simulink model "RefModel_Task"  (R2020a)
settings: Solver=ode1  StartTime=0.0  StopTime=10.0  FixedStep=Ts_Task.Ts_base  RelTol=1e-3
undefined symbols (not defined in the file or in its folder): groundspeedCmd, heightCmd, rollCmd
(part 2 of 5)

== stateflow chart RefModel_Task/Task_StateFlow ==
  state LogData [parallel]
    en:
    settings: executionOrder=17
    state Work
      en,du:
      du_func;
    (default) -> LogData.Work
  state ParserInput [parallel]
    en:
    initPathModeOut;
    initWindParam;
    updateInput;
    enterNum_Land = 0;
    du:
    % ComFlightOut = updateInput;
    updateInput;
    updatePathModeOut;
    % 计算有效航路点数
    PathModeOut.validPathNum = calValidPointNum;
    % 姿态是否稳定
    isAttitudeStable_globalvar = isAttitudeStable;
    % 更新当前航点
    updatePreAndCurPathPoint;
    % on every(300, tick): isPathDataValid;
    settings: executionOrder=1
  state ParserCmd [parallel]
    % 处理Mavlink指令
    en:
    printComInfo('TaskModel Start!!!!',0)
    initInputCmdParam
    du:
    du_func_cmd;
    du_func_singleMode;
    settings: executionOrder=2
    state REMOTE [parallel]
      settings: executionOrder=1
      state Manual
        en:
        manual_du_func
      state Auto
        en:
        auto_du_func
      (default) -> Manual
      Manual -> Auto [order 1] : [IN_MAV.remote_control_t.chG_Mag < 1500]
      Manual -> Auto [order 2] : [TaskParam.getOutOfRemote]
      Auto -> Manual : [IN_MAV.remote_control_t.chG_Mag >= 1500 && ...
          | ~TaskParam.getOutOfRemote]
  state BreakPoint [parallel]
    settings: executionOrder=18
    state BeforePath
      en,du:
    state InPath
      en,du:
    state PauseInPath
      en,du:
    state InGoHome
      en:
      en_func;
    (default) -> BeforePath
    (junction 2115) -> BeforePath
    (junction 2112) -> (junction 2115)
    BeforePath -> InPath : [PathModeOut.flightTaskMode == ENUM_FlightTaskMode.PathFollowMode]
    InPath -> PauseInPath [order 2] : [PathModeOut.flightTaskMode == ENUM_FlightTaskMode.AirStandByMode]
    PauseInPath -> InPath [order 1] : [PathModeOut.flightTaskMode == ENUM_FlightTaskMode.PathFollowMode]
    InPath -> (junction 2121) [order 1]
    PauseInPath -> (junction 2124) [order 2]
    (junction 2124) -> (junction 2121)
    (junction 2121) -> InGoHome : [PathModeOut.flightTaskMode == ENUM_FlightTaskMode.GoHomeMode || ...
        | PathModeOut.flightTaskMode == ENUM_FlightTaskMode.Fix2Rotor_Mode]
    InGoHome -> (junction 2112) : [PathModeOut.flightTaskMode == ENUM_FlightTaskMode.GroundStandByMode]
  state PowerConsumer [parallel]
    settings: executionOrder=3
    state Work
      en,du:
      du_func;
    (default) -> PowerConsumer.Work
  state PrintfCriticalInfo [parallel]
    on every(120,tick): info_60tick();
    settings: executionOrder=4
  state FLIGHTMODE [parallel]
    settings: executionOrder=5
    state AUTO_TASK
      en:
      % 进入模式
      printDebugInfo('AUTOTASK','Enter',1)
      RTInfo.Task = ENUM_RTInfo_Task.Enter_AutoMode; % 更新RT信息
      isAutoMode_globalvar = true;
      PathModeOut.AutoManualMode = ENUM_ControlMode.Auto;
      du:
      du_AUTO_TASK_func;
      ex:
      % 退出模式
      printDebugInfo('AUTOTASK','Exit',1)
      state INIT
        en:
        % 进入模式
        printDebugInfo('INIT','Enter')
        RTInfo.Task = ENUM_RTInfo_Task.Enter_AutoMode_Init; % 更新RT信息
        sendEventWhileEnterAuto
        ex:
        % 退出模式
        printDebugInfo('INIT','Exit')
      state MODE_GOURNDSTANDBY
        en:
        % 进入模式
        printDebugInfo('GroundStandBy','Enter')
        RTInfo.Task = ENUM_RTInfo_Task.Enter_AutoMode_GroundStandBy; % 更新RT信息
        updateLogDataBuffer(ENUM_TaskLogBlockName.TASKLOG_FlightMode,RTInfo.Task,'write'); % 更新log缓存
        PathModeOut.whereIsUAV = ENUM_Where.OnGround;
        hasTaskStarted_globalbar = false;
        ex:
        % 退出模式
        printDebugInfo('GroundStandBy','Exit')
        preTaskMode = ENUM_FlightTaskMode.GroundStandByMode;
        PathModeOut.numTakeOff = PathModeOut.numTakeOff + 1;
        state INIT
          en:
          RTInfo.Task = ENUM_RTInfo_Task.Enter_AutoMode_GroundStandBy_Init; % 更新RT信息
          updateLogDataBuffer(ENUM_TaskLogBlockName.TASKLOG_FlightMode,RTInfo.Task,'write'); % 更新log缓存
          PathModeOut.uavMode = TaskParam.uavMode_InGroundStandByMode;
          PathModeOut.flightTaskMode = ENUM_FlightTaskMode.GroundStandByMode;
          if ~hasTakeOff %  起飞前的地面怠速
          PathModeOut.flightControlMode = ENUM_FlightControlMode.GroundStandByControlMode;
          else % 降落后发动机关车
          PathModeOut.flightControlMode = ENUM_FlightControlMode.RotorShutDown;
          end
          du:
        state TOGO
          en:
          printDebugInfo('GroundStandBy','ToGo')
          RTInfo.Task = ENUM_RTInfo_Task.Enter_AutoMode_GroundStandBy_ToGo; % 更新RT信息
          updateLogDataBuffer(ENUM_TaskLogBlockName.TASKLOG_FlightMode,RTInfo.Task,'write'); % 更新log缓存
          PathModeOut.headingCmd = double(ComFlightOut.curEuler(1));
          du:
          % 实时更新当前航向，避免航向测量修正对起飞模式控制的影响
          PathModeOut.groundspeedCmd = 0;
          % PathModeOut.turnRadiusCmd = 0;
          PathModeOut.heightCmd = 0;
          % 设置侧偏距为0
          PathModeOut.dz = 0;
          % 设置预置滚转
          PathModeOut.rollCmd = 0;
          % 悬停位置
          PathModeOut.turnCenterLL = ComFlightOut.curLLA(1:2);
        (default) -> FLIGHTMODE.AUTO_TASK.MODE_GOURNDSTANDBY.INIT
        FLIGHTMODE.AUTO_TASK.MODE_GOURNDSTANDBY.INIT -> FLIGHTMODE.AUTO_TASK.MODE_GOURNDSTANDBY.TOGO : [isReadyToGo]
      state MODE_TAKEOFF
        en:
        % 进入模式
        printDebugInfo('TakeOff','Enter')
        RTInfo.Task = ENUM_RTInfo_Task.Enter_AutoMode_TakeOff; % 更新RT信息
        updateLogDataBuffer(ENUM_TaskLogBlockName.TASKLOG_FlightMode,RTInfo.Task,'write'); % 更新log缓存
        PathModeOut.whereIsUAV = ENUM_Where.InTheAir;
        hasTakeOff = true;
        du:
        ex:
        % 退出模式
        printDebugInfo('TakeOff','Exit')
        preTaskMode = ENUM_FlightTaskMode.TakeOffMode;
        state INIT
          en:
          RTInfo.Task = ENUM_RTInfo_Task.Enter_AutoMode_TakeOff_Init; % 更新RT信息
          updateLogDataBuffer(ENUM_TaskLogBlockName.TASKLOG_FlightMode,RTInfo.Task,'write'); % 更新log缓存
          PathModeOut.uavMode = TaskParam.uavMode_InTakeOffMode;
          PathModeOut.flightTaskMode = ENUM_FlightTaskMode.TakeOffMode;
          PathModeOut.flightControlMode = ENUM_FlightControlMode.RotorGoUpDownBySpeed;
          % 需计算指令： 高度 航向 速度
          tempIdx = idxStartPathPoint;
          if isPathDataValid && PathModeOut.typeAutoMode == ENUM_AutoModeType.AutoProfile
          % 自动任务模式下
          printDebugInfo('TakeOff','AutoProfile Yes')
          % 航向捕获当前航向
          PathModeOut.headingCmd = double(ComFlightOut.curEuler(1));
          else
          printDebugInfo('TakeOff','AutoProfile No')
          % 航向捕获当前航向
          PathModeOut.headingCmd = double(ComFlightOut.curEuler(1));
          end
          PathModeOut.groundspeedCmd = TaskParam.cruiseSpeed_rotorMode;
          % 设置侧偏距为0
          PathModeOut.dz = 0;
          % 设置预置滚转
          PathModeOut.rollCmd = 0;
          % 悬停位置
          PathModeOut.turnCenterLL = ComFlightOut.curLLA(1:2);
        state DOING_NearGround
          en:
          printDebugInfo('TakeOff','NearGround')
          RTInfo.Task = ENUM_RTInfo_Task.Enter_AutoMode_TakeOff_NearGround; % 更新RT信息
          updateLogDataBuffer(ENUM_TaskLogBlockName.TASKLOG_FlightMode,RTInfo.Task,'write'); % 更新log缓存
          PathModeOut.flightControlMode = ENUM_FlightControlMode.RotorGoUpDownBySpeed;
          PathModeOut.heightCmd = TaskParam.midHeight_TakeOffandLand;
          PathModeOut.maxClimbSpeed = TaskParam.maxClimbSpeed_nearGround_TakeOffandLand;
        state WAITING
          en:
          printDebugInfo('TakeOff','Waiting')
          RTInfo.Task = ENUM_RTInfo_Task.Enter_AutoMode_TakeOff_Waiting; % 更新RT信息
          updateLogDataBuffer(ENUM_TaskLogBlockName.TASKLOG_FlightMode,RTInfo.Task,'write'); % 更新log缓存
          PathModeOut.flightControlMode = ENUM_FlightControlMode.SpotHoverMode;
          PathModeOut.heightCmd = TaskParam.midHeight_TakeOffandLand;
        state DOING_FarGround
          en:
          printDebugInfo('TakeOff','FarGround')
          RTInfo.Task = ENUM_RTInfo_Task.Enter_AutoMode_TakeOff_FarGround; % 更新RT信息
          updateLogDataBuffer(ENUM_TaskLogBlockName.TASKLOG_FlightMode,RTInfo.Task,'write'); % 更新log缓存
          PathModeOut.flightControlMode = ENUM_FlightControlMode.RotorGoUpDownBySpeed;
          PathModeOut.heightCmd = CmdParam_altitude;
          PathModeOut.maxClimbSpeed = TaskParam.maxClimbSpeed_normal_TakeOffandLand+0.5;
        state TOGO
          en:
          printDebugInfo('TakeOff','ToGo')
          RTInfo.Task = ENUM_RTInfo_Task.Enter_AutoMode_TakeOff_ToGo; % 更新RT信息
          updateLogDataBuffer(ENUM_TaskLogBlockName.TASKLOG_FlightMode,RTInfo.Task,'write'); % 更新log缓存
          du:
          % 无条件转入后续模式
          headingMode = 1;
          nextMode = ENUM_FlightTaskMode.Rotor2Fix_Mode ;
          SendEvent_autoGoToNextMode
        state StopHere
          en:
          printDebugInfo('TakeOff','StopHere')
          RTInfo.Task = ENUM_RTInfo_Task.SingleMode_TakeOff_StopHere; % 更新RT信息
          updateLogDataBuffer(ENUM_TaskLogBlockName.TASKLOG_FlightMode,RTInfo.Task,'write'); % 更新log缓存
          du:
        (default) -> FLIGHTMODE.AUTO_TASK.MODE_TAKEOFF.INIT
        FLIGHTMODE.AUTO_TASK.MODE_TAKEOFF.INIT -> (junction 1490)
        (junction 1490) -> DOING_NearGround [order 1] : [hasTaskStarted_globalbar == false]% && ...
            | %ComFlightOut.curLLA(3)<AlgoParams.midHeight_TakeOffandLand+10]
        (junction 1490) -> DOING_FarGround [order 2]
        DOING_NearGround -> WAITING : [hasReachHeight(2)  && isAttitudeStable_globalvar]
        WAITING -> DOING_FarGround : event_startTaskFromAir
            | {hasTaskStarted_globalbar = true;}
        DOING_FarGround -> (junction 2190)
        (junction 2190) -> (junction 2193) [order 1] : [isSingleModeRun]
        (junction 2193) -> FLIGHTMODE.AUTO_TASK.MODE_TAKEOFF.StopHere
        (junction 2190) -> FLIGHTMODE.AUTO_TASK.MODE_TAKEOFF.TOGO [order 2] : [hasReachHeight(2)  && isAttitudeStable_Alevel && after(3,sec) || ...
            | hasReachHeight(5)  && after(5,sec)]
      state MODE_HOVERADJUST
        en:
        % 进入模式
        printDebugInfo('HoverAdjust','Enter')
        HeightCmdBeforeAirStandBy = PathModeOut.heightCmd;
        TaskModeBeforeAirStandBy = preTaskMode;
        HeadingCmdBeforeAirStandBy = PathModeOut.headingCmd;
        PathModeOut.whereIsUAV = ENUM_Where.InTheAir;
        on event_homeChanged: % 着陆过程中暂停时,若home点改变，则继续任务时先gohome
        if (preTaskMode == ENUM_FlightTaskMode.LandMode)  && ...
        PathModeOut.typeAutoMode == ENUM_AutoModeType.SuspendTaskToLand;
        TaskModeBeforeAirStandBy = ENUM_FlightTaskMode.GoHomeMode;
        PathModeOut.typeAutoMode = ENUM_AutoModeType.SuspendTaskToHomeThenLand;
        end
        ex:
        % 退出模式
        printDebugInfo('HoverAdjust','Exit')
        state INIT
          en:
          en_func;
        state WORK
          state DOING
            en:
            en_func;
            du:
            responseManualMove;
          state TOGO
            en:
            printDebugInfo('HoverAdjust','ToGo')
            RTInfo.Task = ENUM_RTInfo_Task.Enter_AutoMode_HoverAdjust_ToGo; % 更新RT信息
            updateLogDataBuffer(ENUM_TaskLogBlockName.TASKLOG_FlightMode,RTInfo.Task,'write'); % 更新log缓存
            switch PathModeOut.typeAutoMode
            case ENUM_AutoModeType.AutoProfile
            RTInfo.Task = ENUM_RTInfo_Task.If_AutoMode_HoverAdjust_ToGo_AutoProfile_Yes; % 更新RT信息
            updateLogDataBuffer(ENUM_TaskLogBlockName.TASKLOG_FlightMode,RTInfo.Task,'write'); % 更新log缓存
            SendEvent_autoGoToNextMode
            case  {ENUM_AutoModeType.SuspendTaskToLand,...
            ENUM_AutoModeType.Fix2Rotor2Home2Land}
            nextMode = ENUM_FlightTaskMode.LandMode;
            SendEvent_autoGoToNextMode
            case ENUM_AutoModeType.SuspendTaskToHome
            case ENUM_AutoModeType.Fix2Rotor2HoverAdjust
            case ENUM_AutoModeType.SuspendTaskToHomeThenLand
            nextMode = ENUM_FlightTaskMode.LandMode;
            SendEvent_autoGoToNextMode
            case ENUM_AutoModeType.PauseInAir
            PathModeOut.typeAutoMode = typeAutoModePre;
            send(event_gotoWaitForContinue,FLIGHTMODE.AUTO_TASK)
            otherwise
            % 保持在当前模式
            end
            du:
            responseManualMove;
          state WaitForContinue
            en:
            printDebugInfo('HoverAdjust','WaitForContinue')
            RTInfo.Task = ENUM_RTInfo_Task.Enter_AutoMode_HoverAdjust_WaitForContinue; % 更新RT信息
            updateLogDataBuffer(ENUM_TaskLogBlockName.TASKLOG_FlightMode,RTInfo.Task,'write'); % 更新log缓存
            du:
            responseManualMove;
          FLIGHTMODE.AUTO_TASK.MODE_HOVERADJUST.WORK.DOING -> (junction 1747) [order 2] : event_gotoWaitForContinue
          FLIGHTMODE.AUTO_TASK.MODE_HOVERADJUST.WORK.DOING -> FLIGHTMODE.AUTO_TASK.MODE_HOVERADJUST.WORK.TOGO [order 1] : [(hasMatchAllConditons && isAttitudeStable_globalvar && after(ceil(6/Ts),tick) && nextMode ~= ENUM_FlightTaskMode.LandMode) || ...
              | (hasReachLatLon_assign(10) && hasReachHeight && isAttitudeStable_globalvar &&  after(ceil(30/Ts),tick) && nextMode ~= ENUM_FlightTaskMode.LandMode) || ...
              | (hasReachLatLon_assign(2) && hasReachHeight && isAttitudeStable_Alevel && after(ceil(6/Ts),tick) && nextMode == ENUM_FlightTaskMode.LandMode) || ...
              | (isAttitudeStable_globalvar && after(ceil(4/Ts),tick) && PathModeOut.typeAutoMode == ENUM_AutoModeType.SuspendTaskToLand)]
          FLIGHTMODE.AUTO_TASK.MODE_HOVERADJUST.WORK.TOGO -> WaitForContinue : event_gotoWaitForContinue
          (junction 1747) -> WaitForContinue
        state StopHere
          en:
          printDebugInfo('HovverAdjust','StopHere')
          RTInfo.Task = ENUM_RTInfo_Task.SingleMode_HovverAdjust_StopHere; % 更新RT信息
          updateLogDataBuffer(ENUM_TaskLogBlockName.TASKLOG_FlightMode,RTInfo.Task,'write'); % 更新log缓存
          du:
        state ExitFromContinue
          en:
          printDebugInfo('HoverAdjust','Enter ExitFromContinue')
          RTInfo.Task = ENUM_RTInfo_Task.Enter_AutoMode_HoverAdjust_ExitFromContinue; % 更新RT信息
          updateLogDataBuffer(ENUM_TaskLogBlockName.TASKLOG_FlightMode,RTInfo.Task,'write'); % 更新log缓存
          SendEvent_ContinueFromPause
          du:
          SendEvent_ContinueFromPause
        (default) -> FLIGHTMODE.AUTO_TASK.MODE_HOVERADJUST.INIT
        FLIGHTMODE.AUTO_TASK.MODE_HOVERADJUST.INIT -> FLIGHTMODE.AUTO_TASK.MODE_HOVERADJUST.WORK.DOING : [isReadyToGo]
        WaitForContinue -> (junction 2199)
        (junction 2199) -> (junction 2197) [order 1] : [isSingleModeRun]
        (junction 2199) -> FLIGHTMODE.AUTO_TASK.MODE_HOVERADJUST.ExitFromContinue [order 2] : manual_continueProfile || ...
            | event_startTaskFromAir % 起飞前半段
        (junction 2197) -> FLIGHTMODE.AUTO_TASK.MODE_HOVERADJUST.StopHere
      state MODE_ROTOR2FIX
        en:
        % 进入模式
        printDebugInfo('Rotor2Fix','Enter')
        RTInfo.Task = ENUM_RTInfo_Task.Enter_AutoMode_Rotor2Fix; % 更新RT信息
        updateLogDataBuffer(ENUM_TaskLogBlockName.TASKLOG_FlightMode,RTInfo.Task,'write'); % 更新log缓存
        PathModeOut.whereIsUAV = ENUM_Where.InTheAir;
        ex:
        % 退出模式
        printDebugInfo('Rotor2Fix','Exit')
        preTaskMode = ENUM_FlightTaskMode.Rotor2Fix_Mode;
        % PathModeOut.uavMode = ENUM_UAVMode.Fix; % 防止该模
        state INIT
          en:
          printDebugInfo('Rotor2Fix','Init')
          RTInfo.Task = ENUM_RTInfo_Task.Enter_AutoMode_Rotor2Fix_Init; % 更新RT信息
          updateLogDataBuffer(ENUM_TaskLogBlockName.TASKLOG_FlightMode,RTInfo.Task,'write'); % 更新log缓存
          PathModeOut.uavMode = TaskParam.uavMode_InRotor2FixMode;
          PathModeOut.flightTaskMode = ENUM_FlightTaskMode.Rotor2Fix_Mode;
          PathModeOut.flightControlMode = ENUM_FlightControlMode.HeightKeepMode;
          % 需计算指令： 高度 航向 速度
          tempIdx = idxStartPathPoint;
          if isPathDataValid && PathModeOut.typeAutoMode == ENUM_AutoModeType.AutoProfile
          printDebugInfo('Rotor2Fix','AutoProfile Yes')
          RTInfo.Task = ENUM_RTInfo_Task.If_AutoMode_Rotor2Fix_Init_AutoProfile_Yes; % 更新RT信息
          updateLogDataBuffer(ENUM_TaskLogBlockName.TASKLOG_FlightMode,RTInfo.Task,'write'); % 更新log缓存
          % 自动任务模式下
          % 高度指令延续前一模式
          % 航向指令延续前一模式
          PathModeOut.groundspeedCmd = TaskParam.cruiseSpeed_cruise;
          else
          printDebugInfo('Rotor2Fix','AutoProfile No')
          % 手动选择该模式
          % 捕获当前高度
          PathModeOut.heightCmd = double(ComFlightOut.curLLA(3));
          % 捕获当前速度,设定最小值
          PathModeOut.groundspeedCmd = max(TaskParam.cruiseSpeed_cruise,ComFlightOut.curGroundSpeed);
          end
          % 捕获当前航向
          PathModeOut.headingCmd = double(ComFlightOut.curEuler(1));
          % 设置侧偏距为0
          PathModeOut.dz = 0;
          % 设置预置滚转
          PathModeOut.rollCmd = 0;
          % 最大爬升率
          PathModeOut.maxClimbSpeed = TaskParam.maxClimbSpeed_fixMode;
        state TOGO
          en:
          printDebugInfo('Rotor2Fix','ToGo')
          RTInfo.Task = ENUM_RTInfo_Task.Enter_AutoMode_Rotor2Fix_ToGo; % 更新RT信息
          updateLogDataBuffer(ENUM_TaskLogBlockName.TASKLOG_FlightMode,RTInfo.Task,'write'); % 更新log缓存
          PathModeOut.uavMode = ENUM_UAVMode.Fix;
          du:
          switch PathModeOut.typeAutoMode
          case ENUM_AutoModeType.AutoProfile
          printDebugInfo('Rotor2Fix','Switch AutoProfile')
          RTInfo.Task = ENUM_RTInfo_Task.If_AutoMode_Rotor2Fix_ToGo_AutoProfile_Yes; % 更新RT信息
          updateLogDataBuffer(ENUM_TaskLogBlockName.TASKLOG_FlightMode,RTInfo.Task,'write'); % 更新log缓存
          SendEvent_autoGoToNextMode
          case {ENUM_AutoModeType.SuspendTaskToHomeThenLand,ENUM_AutoModeType.SuspendTaskToHome}
          printDebugInfo('Rotor2Fix','Switch Fix2Rotor2Home2Land')
          RTInfo.Task = ENUM_RTInfo_Task.If_AutoMode_Rotor2Fix_ToGo_Fix2Rotor2Home2Land_Yes; % 更新RT信息
          updateLogDataBuffer(ENUM_TaskLogBlockName.TASKLOG_FlightMode,RTInfo.Task,'write'); % 更新log缓存
          send(event_fix2Rotor2Home2Land,FLIGHTMODE.AUTO_TASK);
          case ENUM_AutoModeType.SuspendTaskToLand
          printDebugInfo('Rotor2Fix','Switch SuspendTaskToLand')
          RTInfo.Task = ENUM_RTInfo_Task.If_AutoMode_Rotor2Fix_ToGo_SuspendTaskToLand_Yes; % 更新RT信息
          updateLogDataBuffer(ENUM_TaskLogBlockName.TASKLOG_FlightMode,RTInfo.Task,'write'); % 更新log缓存
          send(event_land_GScommand,FLIGHTMODE.AUTO_TASK);
          case ENUM_AutoModeType.Fix2Rotor2HoverAdjust
          printDebugInfo('Rotor2Fix','Switch Fix2Rotor2HoverAdjust')
          RTInfo.Task = ENUM_RTInfo_Task.If_AutoMode_Rotor2Fix_ToGo_Fix2Rotor2HoverAdjust_Yes; % 更新RT信息
          updateLogDataBuffer(ENUM_TaskLogBlockName.TASKLOG_FlightMode,RTInfo.Task,'write'); % 更新log缓存
          send(manual_fix2Rotor,FLIGHTMODE.AUTO_TASK);
          otherwise
          % 保持在当前模式
          end
        state DOING
          en:
          printDebugInfo('Rotor2Fix','Doing')
          RTInfo.Task = ENUM_RTInfo_Task.Enter_AutoMode_Rotor2Fix_Doing; % 更新RT信息
          updateLogDataBuffer(ENUM_TaskLogBlockName.TASKLOG_FlightMode,RTInfo.Task,'write'); % 更新log缓存
          du:
          % 不响应指令高度改变
        state ToHome
          en:
          printDebugInfo('Rotor2Fix','FailToGo')
          RTInfo.Task = ENUM_RTInfo_Task.Rotor2Fix_FailToGo; % 更新RT信息
          updateLogDataBuffer(ENUM_TaskLogBlockName.TASKLOG_FlightMode,RTInfo.Task,'write'); % 更新log缓存
          send(event_fix2Rotor2Home2Land,FLIGHTMODE.AUTO_TASK);
        state StopHere
          en:
          printDebugInfo('Rotor2Fix','StopHere')
          RTInfo.Task = ENUM_RTInfo_Task.SingleMode_Rotor2Fix_StopHere; % 更新RT信息
          updateLogDataBuffer(ENUM_TaskLogBlockName.TASKLOG_FlightMode,RTInfo.Task,'write'); % 更新log缓存
          du:
          state ToGo
            en:
            send(manual_fix2Rotor,FLIGHTMODE.AUTO_TASK);
          state Enter
            en:
          (default) -> Enter
          Enter -> ToGo : after(10,sec)
        (default) -> FLIGHTMODE.AUTO_TASK.MODE_ROTOR2FIX.INIT
        FLIGHTMODE.AUTO_TASK.MODE_ROTOR2FIX.INIT -> FLIGHTMODE.AUTO_TASK.MODE_ROTOR2FIX.DOING
        FLIGHTMODE.AUTO_TASK.MODE_ROTOR2FIX.DOING -> (junction 1156)
        (junction 1156) -> ToHome [order 1] : after(ceil(15/Ts),tick)
        (junction 1156) -> FLIGHTMODE.AUTO_TASK.MODE_ROTOR2FIX.TOGO [order 2] : [hasReachExpectSpeed(14,0) && isAttitudeStable_globalvar && after(ceil(14/Ts),tick)  || ...
            |  hasReachExpectSpeed(18,3) && isAttitudeStable_globalvar && after(ceil(8/Ts),tick)  || ...
            |  hasReachExpectSpeed(20,5) && isAttitudeStable_globalvar && after(ceil(6/Ts),tick)]
            | {printComInfo('Exit Rotor2Fix:Airspeed is %.0f',1,ComFlightOut.curAirSpeed);
            |  printComInfo('Exit Rotor2Fix:Groundspeed is %.0f',1,ComFlightOut.curGroundSpeed);
            | RTInfo.Task = ENUM_RTInfo_Task.Flag_Rotor2Fix_MatchCondition_To_Finish; % 更新RT信息
            |         updateLogDataBuffer(ENUM_TaskLogBlockName.TASKLOG_FlightMode,RTInfo.Task,'write'); % 更新log缓存
            | }
        (junction 1156) -> (junction 2213) [order 3]
        (junction 2213) -> FLIGHTMODE.AUTO_TASK.MODE_ROTOR2FIX.StopHere : [isSingleModeRun]
      state MODE_HOVERUP
        en:
        % 进入模式
        printDebugInfo('HoverUp','Enter')
        RTInfo.Task = ENUM_RTInfo_Task.Enter_AutoMode_HoverUp; % 更新RT信息
        updateLogDataBuffer(ENUM_TaskLogBlockName.TASKLOG_FlightMode,RTInfo.Task,'write'); % 更新log缓存
        PathModeOut.whereIsUAV = ENUM_Where.InTheAir;
        ex:
        % 退出模式
        printDebugInfo('HoverUp','Exit')
        preTaskMode = ENUM_FlightTaskMode.HoverUpMode;
        PathModeOut.turnRadiusCmd = TaskParam.turnR; % 还原hoverup模式中可能改变的盘旋半径
        state INIT_InitialHeight
          en:
          PathModeOut.uavMode = TaskParam.uavMode_InHoverUpDownMode;
          PathModeOut.flightTaskMode = ENUM_FlightTaskMode.HoverUpMode;
          PathModeOut.flightControlMode = ENUM_FlightControlMode.CircleHoverMode;
          if isSingleModeRun
          en_func_HoverUp_SingleMode;
          else
          en_func_HoverUp;
          end
          du:
          updateTurnR_HoverUp();
        state INIT_FinalHeight
          en:
          PathModeOut.heightCmd = double(IN_MAV.mavlink_mission_item_def(1).z);
          du:
          updateTurnR_HoverUp();
        state DOING
          en:
          printDebugInfo('HoverUp','Doing')
          RTInfo.Task = ...
          ENUM_RTInfo_Task.Enter_AutoMode_HoverUp_Doing; % 更新RT信息
          updateLogDataBuffer(ENUM_TaskLogBlockName.TASKLOG_FlightMode,RTInfo.Task,'write'); % 更新log缓存
          du:
          updateTurnR_HoverUp();;
          state R0
          state R1
          state R2
          (default) -> (junction 2356)
          (junction 2356) -> (junction 2358) [order 1] : [PathModeOut.turnRadiusCmd >= 120]
          (junction 2356) -> (junction 2349) [order 2] : [PathModeOut.turnRadiusCmd >= 90 && ...
              | PathModeOut.turnRadiusCmd < 120]
          (junction 2356) -> R0 [order 3]
          (junction 2358) -> R2
          (junction 2349) -> R1
          R1 -> R2 : [PathModeOut.turnRadiusCmd >= 120]{record1(120);}
          R0 -> R1 : [PathModeOut.turnRadiusCmd >= 90 && ...
              | PathModeOut.turnRadiusCmd < 120]{record1(90);}
        state LevelAttitude
          en:
          printDebugInfo('HoverUp','LevelAttitude')
          RTInfo.Task = ...
          ENUM_RTInfo_Task.Enter_AutoMode_HoverUp_LevelAttitude; % 更新RT信息
          updateLogDataBuffer(ENUM_TaskLogBlockName.TASKLOG_FlightMode,RTInfo.Task,'write'); % 更新log缓存
          PathModeOut.flightControlMode = ENUM_FlightControlMode.HeadingKeepMode;
          du:
          PathModeOut.rollCmd = 0;
          PathModeOut.dR_turn = 0;
          % 航向捕获当前航向
          PathModeOut.headingCmd = double(ComFlightOut.curEuler(1));
        state StopHere
          en:
          printDebugInfo('HoverUp','StopHere')
          RTInfo.Task = ENUM_RTInfo_Task.SingleMode_HoverUp_StopHere; % 更新RT信息
          updateLogDataBuffer(ENUM_TaskLogBlockName.TASKLOG_FlightMode,RTInfo.Task,'write'); % 更新log缓存
          du:
        state TOGO
          en:
          printDebugInfo('HoverUp','ToGo')
          du:
          switch PathModeOut.typeAutoMode
          case ENUM_AutoModeType.AutoProfile
          printDebugInfo('HoverUp','Switch AutoProfile')
          RTInfo.Task = ENUM_RTInfo_Task.If_AutoMode_HoverUp_ToGo_AutoProfile_Yes; % 更新RT信息
          updateLogDataBuffer(ENUM_TaskLogBlockName.TASKLOG_FlightMode,RTInfo.Task,'write'); % 更新log缓存
          SendEvent_autoGoToNextMode
          otherwise
          % 保持在当前模式
          end
        (default) -> INIT_InitialHeight
        INIT_InitialHeight -> INIT_FinalHeight : after(5,sec)
        INIT_FinalHeight -> (junction 1060)
        (junction 1060) -> FLIGHTMODE.AUTO_TASK.MODE_HOVERUP.DOING [order 1] : [~hasReachExpectedHeightRange]
        (junction 1060) -> (junction 1057) [order 2] : [hasReachExpectedHeightRange]
        FLIGHTMODE.AUTO_TASK.MODE_HOVERUP.DOING -> (junction 1057) : [hasReachExpectedHeight && ...
            | isHeadingToTarget]
        (junction 1057) -> FLIGHTMODE.AUTO_TASK.MODE_HOVERUP.LevelAttitude
        FLIGHTMODE.AUTO_TASK.MODE_HOVERUP.LevelAttitude -> (junction 2231) : after(0.5,sec)
        (junction 2231) -> (junction 2235) [order 1] : [isSingleModeRun]
        (junction 2235) -> FLIGHTMODE.AUTO_TASK.MODE_HOVERUP.StopHere
        (junction 2231) -> FLIGHTMODE.AUTO_TASK.MODE_HOVERUP.TOGO [order 2]
      state MODE_PATH
        en:
        % 进入模式
        printDebugInfo('PathFollow','Enter')
        PathModeOut.whereIsUAV = ENUM_Where.InTheAir;
        on manual_switchHeight:ResponseEvent_manualSwitchHeight
        ex:
        % 退出模式
        printDebugInfo('PathFollow','Exit')
        preTaskMode = ENUM_FlightTaskMode.PathFollowMode;
        isArrive1stPointInPathMode = false;
        updateLLATaksInterrupt();
        state INIT
          en:
          % 需计算指令： 高度 航向 速度 侧偏距 待飞距离
          en_func;
          ex:
        state ToLastPoint
          en:
          printDebugInfo('PathFollow','ToLastPoint')
          RTInfo.Task = ENUM_RTInfo_Task.Enter_AutoMode_PathFollow_ToLast; % 更新RT信息
          updateLogDataBuffer(ENUM_TaskLogBlockName.TASKLOG_FlightMode,RTInfo.Task,'write'); % 更新log缓存
          tempIdx = PathModeOut.currentPointNum;
          if IN_MAV.mavlink_mission_item_def(tempIdx).param1 ~= 0
          SendEvent_BeginPayLoadWork
          end
          du:
          % 航段起点
          tempIdx = PathModeOut.prePointNum;
          startLLA = double([IN_MAV.mavlink_mission_item_def(tempIdx).x,...
          IN_MAV.mavlink_mission_item_def(tempIdx).y, IN_MAV.mavlink_mission_item_def(tempIdx).z]);
          % 航段终点
          tempIdx = PathModeOut.currentPointNum;
          targetLLA = double([IN_MAV.mavlink_mission_item_def(tempIdx).x,...
          IN_MAV.mavlink_mission_item_def(tempIdx).y, IN_MAV.mavlink_mission_item_def(tempIdx).z]);
          PathModeOut.prePathPoint_LLA = startLLA;
          PathModeOut.curPathPoint_LLA = targetLLA;
          % 更新PathMode输出结构体
          this_mission_item_def = IN_MAV.mavlink_mission_item_def(tempIdx);
          PathModeOut  = updatePathModeStruct(ComFlightOut.curLLA,...
          startLLA,  targetLLA,  PathModeOut,  this_mission_item_def);
          % 侧偏距
          if PathModeOut.validPathNum == 2
          PathModeOut.dz = 0;
          end
          % 处理高度指令
          %if doHeightCmdKeepAfterHeightSwitch
          %    ResponseEvent_manualSwitchHeight
          %end
          % 判断是否到达
          temp_AlgoParams = TaskParam;
          temp_AlgoParams.reachFlag_point_dist = 5;
          arriveFlag = calIfReachPoint_horizontal(ComFlightOut.curLLA,  ...
          startLLA,  targetLLA,  temp_AlgoParams);
          if arriveFlag
          RTInfo.Task = ENUM_RTInfo_Task.If_AutoMode_PathFollow_ToLast_Arrive; % 更新RT信息
          if isDebugInfoToShow
          fprintf('\t\t\t time %.2f [sec]: arrive the %.0fth path point!\n',clock_sec,tempIdx);
          end
          send(event_arrivePoint,FLIGHTMODE.AUTO_TASK.MODE_PATH);
          end
          ex:
          isArrive1stPointInPathMode = true;
          idxTransitPoint = 0;
          SendEvent_StopPayLoadWork
        state ToTheNext
          en:
          printDebugInfo('PathFollow','ToTheNextMode')
          RTInfo.Task = ENUM_RTInfo_Task.Enter_AutoMode_PathFollow_ToLast; % 更新RT信息
          updateLogDataBuffer(ENUM_TaskLogBlockName.TASKLOG_FlightMode,RTInfo.Task,'write'); % 更新log缓存
          du:
          switch PathModeOut.typeAutoMode
          case ENUM_AutoModeType.AutoProfile
          printDebugInfo('PathFollow','Switch AutoProfile')
          RTInfo.Task = ENUM_RTInfo_Task.If_AutoMode_PathFollow_ToGo_AutoProfile_Yes; % 更新RT信息
          updateLogDataBuffer(ENUM_TaskLogBlockName.TASKLOG_FlightMode,RTInfo.Task,'write'); % 更新log缓存
          SendEvent_autoGoToNextMode
          otherwise
          % 保持在当前模式
          printDebugInfo('PathFollow','Switch Otherwise')
          send(manual_airStandBy,FLIGHTMODE.AUTO_TASK);
          end
        state ToFirstPoint
          en:
          printDebugInfo('PathFollow','ToFirstPoint')
          RTInfo.Task = ENUM_RTInfo_Task.Enter_AutoMode_PathFollow_ToFirst; % 更新RT信息
          updateLogDataBuffer(ENUM_TaskLogBlockName.TASKLOG_FlightMode,RTInfo.Task,'write'); % 更新log缓存
          % Debug
          DebugParam.stepNaviPath = 3;
          tempIdx = PathModeOut.currentPointNum;
          if IN_MAV.mavlink_mission_item_def(tempIdx).param1 ~= 0
          SendEvent_BeginPayLoadWork
          end
          % 航段起点
          startLLA = ComFlightOut.curLLA;
          resetPathProgram = true;
          du:
          % Debug
          DebugParam.stepNaviPath = 4;
          du_func
          if PathModeOut.currentPointNum == 2
          du_func_verticalMove
          end
          %
          ex:
          isArrive1stPointInPathMode = true;
          idxTransitPoint = 0;
          resetPathProgram =true;
          SendEvent_StopPayLoadWork
        state ToMidPoint
          en:
          printDebugInfo('PathFollow','ToMidPoint')
          RTInfo.Task = ENUM_RTInfo_Task.Enter_AutoMode_PathFollow_ToMid; % 更新RT信息
          updateLogDataBuffer(ENUM_TaskLogBlockName.TASKLOG_FlightMode,RTInfo.Task,'write'); % 更新log缓存
          tempIdx = PathModeOut.currentPointNum;
          if IN_MAV.mavlink_mission_item_def(tempIdx).param1 ~= 0
          printDebugInfo('PathFollow','Camera Yes')
          SendEvent_BeginPayLoadWork
          else
          printDebugInfo('PathFollow','Camera No')
          end
          du:
          calTransitPoints
          % 处理高度指令
          %if doHeightCmdKeepAfterHeightSwitch
          %    ResponseEvent_manualSwitchHeight
          %end
          if arriveFlag
          RTInfo.Task = ENUM_RTInfo_Task.If_AutoMode_PathFollow_ToMid_Arrive; % 更新RT信息
          updateLogDataBuffer(ENUM_TaskLogBlockName.TASKLOG_FlightMode,RTInfo.Task,'write'); % 更新log缓存
          PathModeOut.prePointNum = PathModeOut.prePointNum+1;
          PathModeOut.currentPointNum = PathModeOut.currentPointNum+1;
          if isDebugInfoToShow
          fprintf('\t\t\t time %.2f [sec]: arrive the %.0fth path point!\n',clock_sec,PathModeOut.prePointNum);
          end
          send(event_arrivePoint,FLIGHTMODE.AUTO_TASK.MODE_PATH);
          end
          ex:
          isArrive1stPointInPathMode = true;
          idxTransitPoint = 0;
          SendEvent_StopPayLoadWork
        (default) -> FLIGHTMODE.AUTO_TASK.MODE_PATH.INIT
        (junction 2271) -> (junction 2273)
        (junction 2273) -> FLIGHTMODE.AUTO_TASK.MODE_PATH.INIT
        (junction 2267) -> (junction 2271)
        FLIGHTMODE.AUTO_TASK.MODE_PATH.INIT -> (junction 328) [order 4] : event_finishPath
        (junction 328) -> (junction 1915)
        ToLastPoint -> (junction 1915) : event_arrivePoint
        (junction 1915) -> (junction 2267) [order 2] : {resetPath}
        (junction 1915) -> ToTheNext [order 1] : [isCompleteLoopPath]
            | {updateTaskCompleteFlag();}
        FLIGHTMODE.AUTO_TASK.MODE_PATH.INIT -> ToLastPoint [order 3] : event_goLastPoint
        FLIGHTMODE.AUTO_TASK.MODE_PATH.INIT -> (junction 332) [order 1]
        (junction 337) -> ToLastPoint
        (junction 332) -> (junction 330) : event_goMidPoint
        (junction 94) -> (junction 337) [order 2] : [isNextTheLastPoint]
        FLIGHTMODE.AUTO_TASK.MODE_PATH.INIT -> ToFirstPoint [order 2] : event_goFirstPoint
        ToFirstPoint -> (junction 330) : event_arrivePoint
        (junction 330) -> (junction 94)
        (junction 94) -> ToMidPoint [order 1] : [~isNextTheLastPoint]
        (junction 335) -> (junction 94)
        ToMidPoint -> (junction 335) : event_arrivePoint
      state MODE_GOHOME
        en:
        % 进入模式
        printDebugInfo('GoHome','Enter')
        PathModeOut.whereIsUAV = ENUM_Where.InTheAir;
        ex:
        % 退出模式
        printDebugInfo('GoHome','Exit')
        preTaskMode = ENUM_FlightTaskMode.GoHomeMode;
        state APPROACHING
          en:
          printDebugInfo('GoHome','Approaching')
          RTInfo.Task = ENUM_RTInfo_Task.Enter_AutoMode_GoHome_Init; % 更新RT信息
          updateLogDataBuffer(ENUM_TaskLogBlockName.TASKLOG_FlightMode,RTInfo.Task,'write'); % 更新log缓存
          en_func;
          % 判断是否需要进行垂直高度调整
          du_func_verticalMove;
          du:
          du_func;
        state TOGO
          en:
          printDebugInfo('GoHome','ToGo')
          RTInfo.Task = ENUM_RTInfo_Task.Enter_AutoMode_GoHome_ToGo; % 更新RT信息
          du:
          du_func;
        (default) -> APPROACHING
        APPROACHING -> FLIGHTMODE.AUTO_TASK.MODE_GOHOME.TOGO : event_getNearHome
      state MODE_HOVERDOWN
        en:
        % 进入模式
        printDebugInfo('HoverDown','Enter')
        PathModeOut.whereIsUAV = ENUM_Where.InTheAir;
        ex:
        % 退出模式
        printDebugInfo('HoverDown','Exit')
        preTaskMode = ENUM_FlightTaskMode.HoverDownMode;
        PathModeOut.isAllowedToPause = true;
        state INIT
          en:
          en_func_HoverDown;
        state DOING
          en:
          printDebugInfo('HoverDown','Doing')
          RTInfo.Task = ENUM_RTInfo_Task.Enter_AutoMode_HoverDown_HeightDown; % 更新RT信息
          updateLogDataBuffer(ENUM_TaskLogBlockName.TASKLOG_FlightMode,RTInfo.Task,'write'); % 更新log缓存
          du:
          updateDownMode();
          PathModeOut.dR_turn = calDradiusWhileTurn(PathModeOut.turnRadiusCmd,...
          ComFlightOut.curLLA(1:2)',PathModeOut.turnCenterLL);
        state TEMP
          du:
          updateDownMode();
          PathModeOut.dR_turn = calDradiusWhileTurn(PathModeOut.turnRadiusCmd,...
          ComFlightOut.curLLA(1:2)',PathModeOut.turnCenterLL);
        state FindWind
          en:
          printDebugInfo('HoverDown','FindWind')
          RTInfo.Task = ENUM_RTInfo_Task.Enter_AutoMode_HoverDown_FindWind; % 更新RT信息
          updateLogDataBuffer(ENUM_TaskLogBlockName.TASKLOG_FlightMode,RTInfo.Task,'write'); % 更新log缓存
          du:
          updateDownMode();
          PathModeOut.dR_turn = calDradiusWhileTurn(PathModeOut.turnRadiusCmd,...
          ComFlightOut.curLLA(1:2)',PathModeOut.turnCenterLL);
        state LevelAttitude
          en:
          printDebugInfo('HoverDown','LevelAttitude')
          RTInfo.Task = ENUM_RTInfo_Task.Enter_AutoMode_HoverDown_LevelAttitude; % 更新RT信息
          updateLogDataBuffer(ENUM_TaskLogBlockName.TASKLOG_FlightMode,RTInfo.Task,'write'); % 更新log缓存
          PathModeOut.flightControlMode = ENUM_FlightControlMode.HeadingKeepMode;
          PathModeOut.isAllowedToPause = false;
          du:
          PathModeOut.rollCmd = 0;
          PathModeOut.dR_turn = 0;
          % 航向捕获当前航向
          PathModeOut.headingCmd = double(ComFlightOut.curEuler(1));
        state StraightForward
          en:
          printDebugInfo('HoverDown','StraightForward')
          RTInfo.Task = ENUM_RTInfo_Task.Enter_AutoMode_HoverDown_StraightForward; % 更新RT信息
          updateLogDataBuffer(ENUM_TaskLogBlockName.TASKLOG_FlightMode,RTInfo.Task,'write'); % 更新log缓存
          PathModeOut.flightControlMode = ENUM_FlightControlMode.HeadingKeepMode;
          enterLLA = ComFlightOut.curLLA;
          en,du:
          dist_straightForward = distOfTwoLL(enterLLA(1:2),ComFlightOut.curLLA(1:2));
        state TOGO
          en:
          printDebugInfo('HoverDown','ToGo')
          RTInfo.Task = ENUM_RTInfo_Task.Enter_AutoMode_HoverDown_ToGo; % 更新RT信息
          updateLogDataBuffer(ENUM_TaskLogBlockName.TASKLOG_FlightMode,RTInfo.Task,'write'); % 更新log缓存
          du:
          du_func;
        state ToCenter
          en:
          printDebugInfo('HoverDown','ToCenter')
          RTInfo.Task = ENUM_RTInfo_Task.Enter_AutoMode_HoverDown_ToCenter; % 更新RT信息
          updateLogDataBuffer(ENUM_TaskLogBlockName.TASKLOG_FlightMode,RTInfo.Task,'write'); % 更新log缓存
          PathModeOut.prePathPoint_LLA = ComFlightOut.curLLA;
          PathModeOut.curPathPoint_LLA = ComFlightOut.curHomeLLA;
          en,du:
          dist_toCenter = distOfTwoLL(PathModeOut.curPathPoint_LLA(1:2), ComFlightOut.curLLA(1:2));
          PathModeOut.headingCmd = calHeadingCmd(ComFlightOut.curLLA, PathModeOut.curPathPoint_LLA);
        (default) -> FLIGHTMODE.AUTO_TASK.MODE_HOVERDOWN.INIT
        FLIGHTMODE.AUTO_TASK.MODE_HOVERDOWN.INIT -> FLIGHTMODE.AUTO_TASK.MODE_HOVERDOWN.DOING : [isReadyToGo]
        FLIGHTMODE.AUTO_TASK.MODE_HOVERDOWN.DOING -> TEMP : [hasReachHeight]
        TEMP -> FindWind : after(1,sec)
        FindWind -> FLIGHTMODE.AUTO_TASK.MODE_HOVERDOWN.LevelAttitude : [willSailAgainstWind]
        FLIGHTMODE.AUTO_TASK.MODE_HOVERDOWN.LevelAttitude -> (junction 2080) : [isAttitudeStable_globalvar]
        (junction 2080) -> StraightForward [order 2]
        (junction 2080) -> FLIGHTMODE.AUTO_TASK.MODE_HOVERDOWN.TOGO [order 1] : [~TaskParam.isHoverDownToCenter]
        StraightForward -> ToCenter : [dist_straightForward > 30]
        ToCenter -> FLIGHTMODE.AUTO_TASK.MODE_HOVERDOWN.TOGO : [dist_toCenter<30 ||...
            |  after(50,sec)]
      state MODE_FIX2ROTOR
        en:
        % 进入模式
        printDebugInfo('Fix2Rotor','Enter')
        PathModeOut.whereIsUAV = ENUM_Where.InTheAir;
        ex:
        % 退出模式
        printDebugInfo('Fix2Rotor','Exit')
        preTaskMode = ENUM_FlightTaskMode.Fix2Rotor_Mode;
        PathModeOut.uavMode = ENUM_UAVMode.Rotor;
        state INIT
          en:
          RTInfo.Task = ENUM_RTInfo_Task.Enter_AutoMode_Fix2Rotor_Init; % 更新RT信息
          updateLogDataBuffer(ENUM_TaskLogBlockName.TASKLOG_FlightMode,RTInfo.Task,'write'); % 更新log缓存
          PathModeOut.uavMode = TaskParam.uavMode_InFix2RotorMode;
          PathModeOut.flightTaskMode = ENUM_FlightTaskMode.Fix2Rotor_Mode;
          PathModeOut.flightControlMode = ENUM_FlightControlMode.HeightKeepMode;
          if isSingleModeRun
          en_func_SingleMode;
          else
          en_func;
          end
        state TOGO
          en:
          printDebugInfo('Fix2Rotor','ToGo')
          PathModeOut.uavMode = ENUM_UAVMode.Rotor;
          du:
          switch PathModeOut.typeAutoMode
          case {ENUM_AutoModeType.AutoProfile,...
          ENUM_AutoModeType.SuspendTaskToHomeThenLand,...
          ENUM_AutoModeType.Fix2Rotor2Home2Land}
          printDebugInfo('Fix2Rotor','Switch AutoProfile')
          RTInfo.Task = ENUM_RTInfo_Task.Fix2Rotor_ToGo_Switch_AutoProfile; % 更新RT信息
          updateLogDataBuffer(ENUM_TaskLogBlockName.TASKLOG_FlightMode,...
          RTInfo.Task,'write'); % 更新log缓存
          SendEvent_autoGoToNextMode
          case ENUM_AutoModeType.Fix2Rotor2HoverAdjust
          printDebugInfo('Fix2Rotor','Switch Fix2Rotor2HoverAdjust')
          RTInfo.Task = ENUM_RTInfo_Task.Fix2Rotor_ToGo_Switch_Fix2Rotor2HoverAdjust; % 更新RT信息
          updateLogDataBuffer(ENUM_TaskLogBlockName.TASKLOG_FlightMode,...
          RTInfo.Task,'write'); % 更新log缓存
          SendEvent_GoTo_HoverAdjust
          otherwise
          printDebugInfo('Fix2Rotor','Switch Otherwise')
          RTInfo.Task = ENUM_RTInfo_Task.Fix2Rotor_ToGo_Switch_Otherwise; % 更新RT信息
          updateLogDataBuffer(ENUM_TaskLogBlockName.TASKLOG_FlightMode,...
          RTInfo.Task,'write'); % 更新log缓存
          SendEvent_GoTo_HoverAdjust
          end
          ex:
        state DOING
          en:
          printDebugInfo('Fix2Rotor','Doing')
          RTInfo.Task = ENUM_RTInfo_Task.Enter_AutoMode_Fix2Rotor_Doing; % 更新RT信息
          updateLogDataBuffer(ENUM_TaskLogBlockName.TASKLOG_FlightMode,...
          RTInfo.Task,'write'); % 更新log缓存
          PathModeOut.flightControlMode = ENUM_FlightControlMode.HeightKeepMode;
          du:
          % 不响应高度指令变更
          % on manual_switchHeight:
          % ResponseEvent_manualSwitchHeight
        state StopHere
          en:
          printDebugInfo('Fix2Rotor','StopHere')
          RTInfo.Task = ENUM_RTInfo_Task.SingleMode_Fix2Rotor_StopHere; % 更新RT信息
          updateLogDataBuffer(ENUM_TaskLogBlockName.TASKLOG_FlightMode,RTInfo.Task,'write'); % 更新log缓存
          du:
        (default) -> FLIGHTMODE.AUTO_TASK.MODE_FIX2ROTOR.INIT
        FLIGHTMODE.AUTO_TASK.MODE_FIX2ROTOR.INIT -> FLIGHTMODE.AUTO_TASK.MODE_FIX2ROTOR.DOING : after(1,sec)
        FLIGHTMODE.AUTO_TASK.MODE_FIX2ROTOR.DOING -> (junction 2254) [order 3] : [TaskParam.isHoverDownToCenter && after(2,sec)]
        (junction 2254) -> (junction 2253)
        FLIGHTMODE.AUTO_TASK.MODE_FIX2ROTOR.DOING -> (junction 2253) [order 1] : [after(TaskParam.timeThreshold_Fix2Rotor+2,sec) && ...
            | isAttitudeStable_globalvar]
            | {fprintf('\t time %.3f [sec]: Fix2Rotor end by %.1f sec\n',clock_sec,...
            | TaskParam.timeThreshold_Fix2Rotor+2);
            | RTInfo.Task = ENUM_RTInfo_Task.Fix2Rotor_ToGo_Complete_Con1; % 更新RT信息
            |     updateLogDataBuffer(ENUM_TaskLogBlockName.TASKLOG_FlightMode,...
            |         RTInfo.Task,'write'); % 更新log缓存
            | }
        (junction 2253) -> (junction 2252)
        FLIGHTMODE.AUTO_TASK.MODE_FIX2ROTOR.DOING -> (junction 2252) [order 2] : [hasReachExpectSpeed && isAttitudeStable_Alevel && ...
            |  after(TaskParam.timeThreshold_Fix2Rotor,sec)]
            | {fprintf('\t time %.3f [sec]: Fix2Rotor end by ExpectSpeed\n',clock_sec);
            | RTInfo.Task = ENUM_RTInfo_Task.Fix2Rotor_ToGo_Complete_Con2; % 更新RT信息
            |     updateLogDataBuffer(ENUM_TaskLogBlockName.TASKLOG_FlightMode,...
            |         RTInfo.Task,'write'); % 更新log缓存
            | }
        (junction 2252) -> FLIGHTMODE.AUTO_TASK.MODE_FIX2ROTOR.TOGO [order 2]
        (junction 2252) -> FLIGHTMODE.AUTO_TASK.MODE_FIX2ROTOR.StopHere [order 1] : [isSingleModeRun]
      state MODE_LAND
        en:
        % 进入模式
        printDebugInfo('Land','Enter')
        PathModeOut.whereIsUAV = ENUM_Where.InTheAir;
        enterNum_Land = enterNum_Land + 1;
        du:
        isReadyToLand;
        updateLandMaxHeight;
        ex:
        % 退出模式
        printDebugInfo('Land','Exit')
        preTaskMode = ENUM_FlightTaskMode.LandMode;
        state LandProg [parallel]
          settings: executionOrder=1
          state INIT
            en:
            RTInfo.Task = ENUM_RTInfo_Task.Enter_AutoMode_Land_Init; % 更新RT信息
            updateLogDataBuffer(ENUM_TaskLogBlockName.TASKLOG_FlightMode, RTInfo.Task,'write'); % 更新log缓存
            PathModeOut.uavMode = TaskParam.uavMode_InLandMode;
            PathModeOut.flightTaskMode = ENUM_FlightTaskMode.LandMode;
            PathModeOut.flightControlMode = ENUM_FlightControlMode.RotorGoUpDownBySpeed;
            % 需计算指令： 高度 航向 速度
            tempIdx = idxStartPathPoint;
            if isPathDataValid && PathModeOut.typeAutoMode == ENUM_AutoModeType.AutoProfile
            printDebugInfo('Land','AutoProfile Yes')
            RTInfo.Task = ENUM_RTInfo_Task.If_AutoMode_Land_Init_AutoProfile_Yes; % 更新RT信息
            updateLogDataBuffer(ENUM_TaskLogBlockName.TASKLOG_FlightMode, RTInfo.Task,'write'); % 更新log缓存
            % 自动任务模式下
            % 航向指令延续上一模式
            else
            printDebugInfo('Land','AutoProfile No')
            % 航向捕获当前航向
            PathModeOut.headingCmd = double(ComFlightOut.curEuler(1));
            end
            PathModeOut.heightCmd = TaskParam.midHeight_TakeOffandLand;
            PathModeOut.groundspeedCmd = TaskParam.cruiseSpeed_rotorMode;
            % 设置侧偏距为0
            PathModeOut.dz = 0;
            % 设置预置滚转
            PathModeOut.rollCmd = 0;
            en_func();
          state FarGround
            en:
            printDebugInfo('Land','FarGround')
            RTInfo.Task = ENUM_RTInfo_Task.Enter_AutoMode_Land_FarGround; % 更新RT信息
            updateLogDataBuffer(ENUM_TaskLogBlockName.TASKLOG_FlightMode, RTInfo.Task,'write'); % 更新log缓存
            PathModeOut.heightCmd = TaskParam.midHeight_TakeOffandLand;
            isLatLonOK_Land = false;
            PathModeOut.turnCenterLL = ComFlightOut.curLLA(1:2) + moveLandMark;
            PathModeOut.maxClimbSpeed = TaskParam.maxClimbSpeed_normal_TakeOffandLand;
            % PathModeOut.heightCmd = double(ComFlightOut.curLLA(3));
            du:
            % 将该函数放在du中,是为了能够实时响应Home的变化
            du_func_eval;
          state NearGround
            en:
            printDebugInfo('Land','NearGround')
            RTInfo.Task = ENUM_RTInfo_Task.Enter_AutoMode_Land_NearGround; % 更新RT信息
            updateLogDataBuffer(ENUM_TaskLogBlockName.TASKLOG_FlightMode, ...
            RTInfo.Task,'write'); % 更新log缓存
            PathModeOut.flightControlMode = ENUM_FlightControlMode.RotorGoUpDownBySpeed;
            PathModeOut.heightCmd = TaskParam.heightCmd_FinalLand;
            en_func;
            du:
            % 最大爬升率
            du_update_HeightCmd;
            du_update_VdCmd;
            du_update_Center;
          state Empty
            ex:
            RTInfo.Task = ENUM_RTInfo_Task.If_AutoMode_Land_HasLand_Yes; % 更新RT信息
          state UnLoad
            en:
            printDebugInfo('Land','UnloadOnGround')
            RTInfo.Task = ENUM_RTInfo_Task.Enter_AutoMode_Land_UnloadOnGround; % 更新RT信息
            updateLogDataBuffer(ENUM_TaskLogBlockName.TASKLOG_FlightMode, RTInfo.Task,'write'); % 更新log缓存
            PathModeOut.flightControlMode = ENUM_FlightControlMode.RotorUnloadToStandby;
            % PathModeOut.heightCmd = 0;
            % PathModeOut.maxClimbSpeed = AlgoParams.maxClimbSpeed_nearGround_TakeOffandLand;
          state TOGO
            en:
            printDebugInfo('Land','ToGo')
            RTInfo.Task = ENUM_RTInfo_Task.Enter_AutoMode_Land_ToGo; % 更新RT信息
            updateLogDataBuffer(ENUM_TaskLogBlockName.TASKLOG_FlightMode, RTInfo.Task,'write'); % 更新log缓存
            switch PathModeOut.typeAutoMode
            case ENUM_AutoModeType.AutoProfile
            printDebugInfo('Land','Switch AutoProfile')
            RTInfo.Task = ENUM_RTInfo_Task.If_AutoMode_Land_ToGo_AutoProfile_Yes; % 更新RT信息
            updateLogDataBuffer(ENUM_TaskLogBlockName.TASKLOG_FlightMode, RTInfo.Task,'write'); % 更新log缓存
            otherwise
            printDebugInfo('Land','Switch AutoProfile')
            end
            du:
            switch PathModeOut.typeAutoMode
            case ENUM_AutoModeType.AutoProfile
            SendEvent_autoGoToNextMode
            otherwise
            SendEvent_autoGoToNextMode
            % 保持在当前模式
            end
          (default) -> FLIGHTMODE.AUTO_TASK.MODE_LAND.LandProg.INIT
          FLIGHTMODE.AUTO_TASK.MODE_LAND.LandProg.INIT -> (junction 1957)
          (junction 1957) -> (junction 1958)
          (junction 1958) -> FarGround [order 2]
          (junction 1958) -> (junction 1962) [order 1] : [hasReachNearGroundHeight]
          FarGround -> (junction 2280) [order 2] : [isLandUncondition]
          (junction 2280) -> (junction 2284)
          FarGround -> NearGround [order 1] : [hasReachNearGroundHeight && isLatLonOK_Land && isAttitudeStable_globalvar && after(ceil(2/Ts),tick) || ...
              | hasReachNearGroundHeight && isAttitudeStable_globalvar && PathModeOut.typeAutoMode == ENUM_AutoModeType.SuspendTaskToLand]
          NearGround -> (junction 1495) : [hasLanded]
              | {PathModeOut.whereIsUAV = ENUM_Where.OnGround;}
          (junction 1495) -> Empty
          (junction 2284) -> NearGround
          (junction 1962) -> NearGround
          Empty -> UnLoad : after(1,tick)
          UnLoad -> FLIGHTMODE.AUTO_TASK.MODE_LAND.LandProg.TOGO : after(1,tick)
        state GPSStatus [parallel]
          settings: executionOrder=2
          state Normal
            en:
            PathModeOut.turnCenterLL = ComFlightOut.curLLA(1:2) + moveLandMark;
            printDebugInfo('Land','At least one GPS available')
            RTInfo.Task = ENUM_RTInfo_Task.Land_AtLeastOne_GPS_Available; % 更新RT信息
            updateLogDataBuffer(ENUM_TaskLogBlockName.TASKLOG_FlightMode, RTInfo.Task,'write'); % 更新log缓存
          state Abnormal
            en:
            PathModeOut.flightControlMode = ENUM_FlightControlMode.RotorGoUpDownWithHorizonPosFree;
            printDebugInfo('Land','No GPS available')
            RTInfo.Task = ENUM_RTInfo_Task.Land_No_GPS_Available; % 更新RT信息
            updateLogDataBuffer(ENUM_TaskLogBlockName.TASKLOG_FlightMode, RTInfo.Task,'write'); % 更新log缓存
            du:
            PathModeOut.turnCenterLL = ComFlightOut.curLLA(1:2) + moveLandMark;
          (default) -> FLIGHTMODE.AUTO_TASK.MODE_LAND.GPSStatus.Normal
          FLIGHTMODE.AUTO_TASK.MODE_LAND.GPSStatus.Normal -> Abnormal : [~isAnyGPSOk]
          Abnormal -> FLIGHTMODE.AUTO_TASK.MODE_LAND.GPSStatus.Normal : [isAnyGPSOk]
      state MODE_AIRSTANDBY
        en:
        % 进入模式
        printDebugInfo('AirStandBy','Enter')
        HeightCmdBeforeAirStandBy = PathModeOut.heightCmd;
        TaskModeBeforeAirStandBy = preTaskMode;
        HeadingCmdBeforeAirStandBy = PathModeOut.headingCmd;
        PathModeOut.whereIsUAV = ENUM_Where.InTheAir;
        ex:
        % 退出模式
        PathModeOut.turnRadiusCmd = TaskParam.turnR; % 还原该模式中可能改变的盘旋半径
        printDebugInfo('AirStandBy','Exit')
        state INIT
          en:
          RTInfo.Task = ENUM_RTInfo_Task.Enter_AutoMode_AirStandBy_Init; % 更新RT信息
          updateLogDataBuffer(ENUM_TaskLogBlockName.TASKLOG_FlightMode, RTInfo.Task,'write'); % 更新log缓存
          PathModeOut.uavMode = TaskParam.uavMode_InAirStandByMode;
          PathModeOut.flightTaskMode = ENUM_FlightTaskMode.AirStandByMode;
          PathModeOut.flightControlMode = ENUM_FlightControlMode.CircleHoverMode;
          en_func_AirStandBy
        state DOING
          en:
          printDebugInfo('AirStandBy','Doing')
          RTInfo.Task = ENUM_RTInfo_Task.Enter_AutoMode_AirStandBy_Doing; % 更新RT信息
          updateLogDataBuffer(ENUM_TaskLogBlockName.TASKLOG_FlightMode, RTInfo.Task,'write'); % 更新log缓存
          du:
          if preTaskMode == ENUM_FlightTaskMode.HoverUpMode;
          PathModeOut.turnRadiusCmd = PathModeOut.turnRadiusCmd_HoverUp;
          end
          PathModeOut.dR_turn = calDradiusWhileTurn(PathModeOut.turnRadiusCmd,...
          ComFlightOut.curLLA(1:2)',PathModeOut.turnCenterLL);
          % on manual_switchHeight:ResponseEvent_manualSwitchHeight
        state ExitFromContinue
          en:
          printDebugInfo('AirStandBy','ExitFromContinue')
          RTInfo.Task = ENUM_RTInfo_Task.Enter_AutoMode_AirStandBy_ToGo; % 更新RT信息
          updateLogDataBuffer(ENUM_TaskLogBlockName.TASKLOG_FlightMode, RTInfo.Task,'write'); % 更新log缓存
          du:
          PathModeOut.dR_turn = calDradiusWhileTurn(PathModeOut.turnRadiusCmd,...
          ComFlightOut.curLLA(1:2)',PathModeOut.turnCenterLL);
          if isHeadingToTarget || preTaskMode == ENUM_FlightTaskMode.HoverDownMode ||...
          preTaskMode == ENUM_FlightTaskMode.HoverUpMode
          SendEvent_ContinueFromPause
          end
        (default) -> FLIGHTMODE.AUTO_TASK.MODE_AIRSTANDBY.INIT
        FLIGHTMODE.AUTO_TASK.MODE_AIRSTANDBY.INIT -> FLIGHTMODE.AUTO_TASK.MODE_AIRSTANDBY.DOING : [isReadyToGo]
        FLIGHTMODE.AUTO_TASK.MODE_AIRSTANDBY.DOING -> FLIGHTMODE.AUTO_TASK.MODE_AIRSTANDBY.ExitFromContinue : manual_continueProfile
      state MODE_STALLRECOVERY
        en:
        % 进入模式
        printDebugInfo('StallRecovery','Enter')
        PathModeOut.whereIsUAV = ENUM_Where.InTheAir;
        ex:
        % 退出模式
        printDebugInfo('StallRecovery','Exit')
        RTInfo.Task = ENUM_RTInfo_Task.StallRecovery_Exit; % 更新RT信息
        updateLogDataBuffer(ENUM_TaskLogBlockName.TASKLOG_FlightMode, RTInfo.Task,'write'); % 更新log缓存
        state StablizePitchAndRoll
          en:
          en_func
          du:
          state Stable
            en:
            stableTime0 = clock_sec;
            du:
          state notStable
            en:
          (default) -> Stable
          notStable -> Stable : [isPitchRollStable]
          Stable -> notStable : [~isPitchRollStable]
        state HeightStable
          en:
          PathModeOut.heightCmd = double(ComFlightOut.curLLA(3));
          % 地速
          PathModeOut.groundspeedCmd = 0;
          PathModeOut.flightControlMode = ENUM_FlightControlMode.RotorStable_RollPitchHeight;
          du:
        state HoverKeeping
          en:
          printDebugInfo('StallRecovery','HoverKeeping')
          RTInfo.Task = ENUM_RTInfo_Task.Enter_AutoMode_StallRecovery_Hover; % 更新RT信息
          updateLogDataBuffer(ENUM_TaskLogBlockName.TASKLOG_FlightMode, RTInfo.Task,'write'); % 更新log缓存
          PathModeOut.flightControlMode = ENUM_FlightControlMode.SpotHoverMode;
          % 捕获当前航向
          PathModeOut.headingCmd = double(ComFlightOut.curEuler(1));
          % 捕获当前高度
          PathModeOut.heightCmd = double(ComFlightOut.curLLA(3));
          % 地速
          PathModeOut.groundspeedCmd = 0;
          % 设置侧偏距为0
          PathModeOut.dz = 0;
          % 设置预置滚转
          PathModeOut.rollCmd = 0;
          % 悬停位置
          PathModeOut.turnCenterLL = ComFlightOut.curLLA(1:2);
        state End
          en:
          send(event_goHomeThenLand_StallRecovery,FLIGHTMODE.AUTO_TASK)
        (default) -> StablizePitchAndRoll
        StablizePitchAndRoll -> End [order 2] : after(10,sec)
        StablizePitchAndRoll -> HeightStable [order 1] : [0 && isPitchRollStableLongEnough]
        HeightStable -> HoverKeeping : after(4,sec)
        HoverKeeping -> End : [hasMatchAllConditons || after(4,sec)]
      state MODE_VerticalMove
        en:
        % 进入模式
        printDebugInfo('VerticalMove','Enter')
        PathModeOut.whereIsUAV = ENUM_Where.InTheAir;
        headingIN_VerticalMove = ComFlightOut.curEuler(1);
        ex:
        % 退出模式
        printDebugInfo('VerticalMove','Exit')
        RTInfo.Task = ENUM_RTInfo_Task.VerticalMove_Exit; % 更新RT信息
        updateLogDataBuffer(ENUM_TaskLogBlockName.TASKLOG_FlightMode, RTInfo.Task,'write'); % 更新log缓存
        preTaskMode = ENUM_FlightTaskMode.VerticalMove;
        state VerticalMove
          en:
          en_func();
          du:
          du_func();
        state GoToNext
          en,du:
          du_func();
        (default) -> VerticalMove
        VerticalMove -> (junction 2058) : [reachHeight]
        (junction 2058) -> GoToNext [order 2] : [~isUavInFix]
        (junction 2058) -> GoToNext [order 1] : [isUavInFix && isHeadingToTarget]
      (default) -> FLIGHTMODE.AUTO_TASK.INIT
      AUTO_TASK -> (junction 1722) [order 11] : manual_groundStandBy || event_single_groundMode
      (junction 435) -> (junction 1722) : %{initInputCmdParam;}
      (junction 1722) -> MODE_GOURNDSTANDBY : % {initPathModeOut;}
      (junction 433) -> (junction 435)
      AUTO_TASK -> (junction 2180) [order 19] : event_single_takeOffMode
      (junction 2180) -> (junction 1198)
      AUTO_TASK -> (junction 1198) [order 4] : manual_takeOff || event_startTaskFromAir
          | [isAllowedToEnterThisMode...
          | (ENUM_FlightTaskMode.TakeOffMode)]
      (junction 1198) -> MODE_TAKEOFF : {%initPathModeOut;
          | %PathModeOut.typeAutoMode = ENUM_AutoModeType.AutoProfile;
          | }
      (junction 1200) -> (junction 1198)
      AUTO_TASK -> (junction 1200) [order 13] : manual_rotorGoUp
      (junction 1580) -> (junction 1200)
      MODE_TAKEOFF -> (junction 507) : auto_gotoNextMode
      AUTO_TASK -> (junction 1580) [order 17] : event_startTaskFromAir % 直接通过开始任务按钮起飞
          | [isAllowedToAutoFlight && ...
          | BatteryOut.batteryStatus == ENUM_BatteryStatus.BatteryNormal && ...
          | PathModeOut.flightTaskMode == ENUM_FlightTaskMode.GroundStandByMode && ...
          |  isUavInRotor]
      AUTO_TASK -> (junction 743) [order 20] : event_single_hoverAdjustMode
          | {nextMode = ENUM_FlightTaskMode.Rotor2Fix_Mode;
          | typeAutoModePre = ENUM_AutoModeType.SingleModeRun;}
      (junction 743) -> (junction 507)
      (junction 736) -> (junction 507)
      (junction 2183) -> (junction 743)
      (junction 507) -> MODE_HOVERADJUST
      (junction 1742) -> (junction 736) : {headingMode = 0;nextMode = ENUM_FlightTaskMode.LandMode;}
      AUTO_TASK -> (junction 2183) [order 6] : manual_hoverAdjust
          | [isAllowedToEnterThisMode...
          | (ENUM_FlightTaskMode.HoverAdjustMode)]
          | {headingMode = 0;}
      (junction 1000) -> (junction 2183)
      (junction 1127) -> (junction 1000)
      (junction 1128) -> (junction 1127) [order 2] : %[isUavInRotor]
          | {setCmdWhileEnterHoverAdjustFromAirStandBy}
      (junction 740) -> (junction 1000) [order 2] : % [isUavInRotor || isUavInFix2Rotor]
          | {headingMode = 0;}
      MODE_HOVERADJUST -> (junction 318) : auto_gotoNextMode
      (junction 318) -> MODE_LAND [order 1] : [nextMode == ENUM_FlightTaskMode.LandMode ]
      (junction 318) -> (junction 509) [order 2] : [nextMode == ENUM_FlightTaskMode.Rotor2Fix_Mode ]
      AUTO_TASK -> (junction 2201) [order 9] : manual_rotor2Fix
          | [isAllowedToEnterThisMode...
          | (ENUM_FlightTaskMode.Rotor2Fix_Mode)]
      (junction 2201) -> (junction 509)
      (junction 2203) -> (junction 2201)
      (junction 509) -> MODE_ROTOR2FIX
      AUTO_TASK -> (junction 2203) [order 21] : event_single_rotor2FixMode
      MODE_ROTOR2FIX -> (junction 511) : auto_gotoNextMode
      AUTO_TASK -> (junction 2216) [order 7] : manual_hoverUp
          | [isAllowedToEnterThisMode...
          | (ENUM_FlightTaskMode.HoverUpMode)]
      (junction 2216) -> (junction 511)
      (junction 2215) -> (junction 2216)
      (junction 511) -> MODE_HOVERUP
      AUTO_TASK -> (junction 2215) [order 22] : event_single_hoverUpMode
      MODE_HOVERUP -> (junction 373) : auto_gotoNextMode
      AUTO_TASK -> (junction 2239) [order 3] : manual_goIntoPath
          | [isAllowedToEnterThisMode...
          | (ENUM_FlightTaskMode.PathFollowMode)]
      (junction 2239) -> (junction 373)
      (junction 2238) -> (junction 2239)
      (junction 373) -> MODE_PATH
      AUTO_TASK -> (junction 2238) [order 23] : event_single_pathMode
      MODE_PATH -> MODE_GOHOME : auto_gotoNextMode
      AUTO_TASK -> (junction 1239) [order 14] : event_goHomeThenLand_VeryHighWind || event_oneKeyGoHome || ...
          | event_goHome_ComLost || event_goHome_NotInFense || ...
          | event_goHomeThenLand_TooLowInFix || event_goHomeThenLand_BatteryLow || ...
          | event_goHomeThenLand_StallRecovery || event_goHomeThenLand_SensorDegrade || ...
          | event_goHomeThenLand_AirspeedFalut || event_goHomeThenLand_LargeOffsetInLand
          | [isAllowedToEnterThisMode...
          | (ENUM_FlightTaskMode.GoHomeMode) ] %isInTheAir && (isUavInRotor || isUavInFix)] % PathModeOut.flightTaskMode ~= ENUM_FlightTaskMode.LandMode
          | {PathModeOut.typeAutoMode = ENUM_AutoModeType.SuspendTaskToHomeThenLand;}
      (junction 1239) -> (junction 1237)
      AUTO_TASK -> (junction 1237) [order 5] : manual_goHomePoint
          | [isAllowedToEnterThisMode...
          | (ENUM_FlightTaskMode.GoHomeMode)] % 响应暂停继续
      (junction 1237) -> MODE_GOHOME
      MODE_GOHOME -> (junction 1742) [order 2] : event_directToHoverFromGoHome
          | [isAllowedToEnterThisMode...
          | (ENUM_FlightTaskMode.HoverAdjustMode)]
      (junction 2243) -> (junction 1237)
      (junction 734) -> (junction 1742)
      MODE_FIX2ROTOR -> MODE_GOHOME [order 2] : auto_gotoNextMode
      AUTO_TASK -> (junction 2243) [order 24] : event_single_goHomeMode
      MODE_GOHOME -> MODE_HOVERDOWN [order 1] : auto_gotoNextMode
      AUTO_TASK -> MODE_HOVERDOWN [order 12] : manual_hoverDown
          | [isAllowedToEnterThisMode...
          | (ENUM_FlightTaskMode.HoverDownMode)]
      MODE_HOVERDOWN -> MODE_FIX2ROTOR : auto_gotoNextMode
      AUTO_TASK -> MODE_FIX2ROTOR [order 10] : manual_fix2Rotor
          | [isAllowedToEnterThisMode...
          | (ENUM_FlightTaskMode.Fix2Rotor_Mode)]
          | {PathModeOut.typeAutoMode = ENUM_AutoModeType.Fix2Rotor2HoverAdjust;}
      MODE_FIX2ROTOR -> (junction 734) [order 1] : auto_goto_HoverAdjustMode
      AUTO_TASK -> MODE_FIX2ROTOR [order 16] : event_fix2Rotor2Home2Land || ...
          | event_fix2Rotor2Home2Land_AirspeedFalut
          | [isAllowedToEnterThisMode...
          | (ENUM_FlightTaskMode.Fix2Rotor_Mode)]
          | {PathModeOut.typeAutoMode = ENUM_AutoModeType.Fix2Rotor2Home2Land;}
      (junction 740) -> MODE_FIX2ROTOR [order 1] : [isUavInFix || ...
          | isUavInRotor2Fix]
      (junction 738) -> (junction 740)
      AUTO_TASK -> MODE_LAND [order 8] : manual_land
          | [isAllowedToEnterThisMode...
          | (ENUM_FlightTaskMode.LandMode)]
      MODE_LAND -> (junction 433) : auto_gotoNextMode
      AUTO_TASK -> (junction 1128) [order 2] : manual_airStandBy
          | [PathModeOut.isAllowedToPause && ...
          | isAllowedToEnterThisMode(ENUM_FlightTaskMode.AirStandByMode)]
          | {typeAutoModePre = PathModeOut.typeAutoMode;
          | PathModeOut.typeAutoMode = ENUM_AutoModeType.PauseInAir;}
      (junction 1128) -> MODE_AIRSTANDBY [order 1] : [isUavInFix]
      AUTO_TASK -> (junction 738) [order 1] : event_land_GScommand || ...
          | event_land_SensorNotHealth || ...
          | event_land_BatterySevereLow
          | [isInTheAir && ...
          | PathModeOut.flightTaskMode ~= ENUM_FlightTaskMode.LandMode]
          | {landPosMode = ENUM_LandMode.CurVTL;
          | PathModeOut.typeAutoMode = ENUM_AutoModeType.SuspendTaskToLand;
          | nextMode = ENUM_FlightTaskMode.LandMode;}
      AUTO_TASK -> MODE_STALLRECOVERY [order 15] : event_stallRecovery
          | [isUavInFix && isInTheAir]
      AUTO_TASK -> MODE_VerticalMove [order 18] : event_verticalMove
          | [isInTheAir]
    state MANUAL
      % 手动转自动要求：在地面，或固定翼飞行，或低速空中旋翼飞行
      en:
      % 进入模式
      printDebugInfo('MANUAL','Enter',1)
      RTInfo.Task = ENUM_RTInfo_Task.Enter_ManualMode; % 更新RT信息
      isAutoMode_globalvar = false;
      PathModeOut.AutoManualMode = ENUM_ControlMode.Manual;
      du:
      % 模式运行
      du_func_manual
      ex:
      % 退出模式
      printDebugInfo('MANUAL','Exit',1)
    (default) -> MANUAL : {setFlightModeInitState}
    MANUAL -> AUTO_TASK : [willEnterAutoMode]
    AUTO_TASK -> MANUAL [order 1] : [willEnterManualMode]
  state CalHomeParam [parallel]
    settings: executionOrder=6
    state Lock
      en:
      if isDebugInfoToShow
      fprintf('%.3f sec: Lock\n',clock_sec);
      end
      initHomeParam
      du:
      initHomeParam
    state Unlock
      en:
      if isDebugInfoToShow
      fprintf('%.3f sec: UnLock\n',clock_sec);
      end
      en_func
      du:
    (default) -> (junction 1528) : {initHomeParam}
    (junction 1528) -> Lock [order 2]
    (junction 1528) -> (junction 1527) [order 1] : [IN_OnPlane.unlock]
    Lock -> CalHomeParam.Unlock : [isOnGround && ...
        | IN_OnPlane.unlock]
    CalHomeParam.Unlock -> Lock : [~IN_OnPlane.unlock]
    (junction 1527) -> CalHomeParam.Unlock
  state Payload [parallel]
    settings: executionOrder=7
    state CAMERA [parallel]
      settings: executionOrder=1
      state STANDBY
        en:
        RTInfo.Task = ENUM_RTInfo_Task.TaskLog_Payload_Camera_StandBy; % 更新RT信息
        updateLogDataBuffer(ENUM_TaskLogBlockName.TASKLOG_Payload,RTInfo.Task,'write');
      state WORK
        en:
        RTInfo.Task = ENUM_RTInfo_Task.TaskLog_Payload_Camera_BeginWork; % 更新RT信息
        updateLogDataBuffer(ENUM_TaskLogBlockName.TASKLOG_Payload,RTInfo.Task,'write');
        du:
        % PayloadControlOut.CAMERA.trigger = 0;
        if doTakePicture
        PayloadControlOut.CAMERA.time = clock_sec;
        PayloadControlOut.CAMERA.trigger = PayloadControlOut.CAMERA.trigger + 1;
        PayloadControlOut.CAMERA.LLA = ComFlightOut.curLLA';
        PayloadControlOut.CAMERA.groundspeed = ComFlightOut.curGroundSpeed;
        RTInfo.Task = ENUM_RTInfo_Task.TaskLog_Payload_Camera_Shot; % 更新RT信息
        updateLogDataBuffer(ENUM_TaskLogBlockName.TASKLOG_Payload,RTInfo.Task,'write');
        if isDebugInfoToShow && rem(int16(PayloadControlOut.CAMERA.trigger),10) == 0
        if 1
        fprintf(' \t\t\t\t %.3f sec: Shot %d\n',clock_sec,...
        int16(PayloadControlOut.CAMERA.trigger));
        else
        fprintf(' \t\t\t\t %.3f sec: Shot %d at (%.6f,%.6f,%.1f)\n',clock_sec,...
        int16(PayloadControlOut.CAMERA.trigger),...
        PayloadControlOut.CAMERA.LLA(1),PayloadControlOut.CAMERA.LLA(2),...
        PayloadControlOut.CAMERA.LLA(3));
        end
        end
        end
      (default) -> Payload.CAMERA.STANDBY : {initCameraStruct;}
      Payload.CAMERA.WORK -> Payload.CAMERA.STANDBY : payload_stopWork
      Payload.CAMERA.STANDBY -> Payload.CAMERA.WORK : payload_beginWork
    state LIADAR [parallel]
      settings: executionOrder=2
      state STANDBY
      state WORK
      (default) -> Payload.LIADAR.STANDBY : {PayloadControlOut.LIDAR.trigger = 0;}
      Payload.LIADAR.STANDBY -> Payload.LIADAR.WORK
  state CalOnPlaneStoreData [parallel]
    settings: executionOrder=9
    state Mileage
      state Endurance
        state Moving
          en:
          du:
          on every(30,tick):
          increaseMileage
          on every(500,tick):
          printComInfo('mileage %.0f [m]',2,...
          BatteryOut.mileage)
        state Static
          du:
        Static -> Moving : [isMoving]
        Moving -> Static : [~isMoving]
      (default) -> Static : {initBatteryOut;}
  state UpdateStoreData [parallel]
    settings: executionOrder=8
    state Updating
      en:
      initAllData
      du:
      updataData
    (default) -> Updating
  state CommunicationLost_Protect [parallel]
    settings: executionOrder=12
    state CommunicationNormal
      en:
      RTInfo.Task = ENUM_RTInfo_Task.TaskLog_Protect_Com_Normal;% 更新RTInfo Task
      updateLogDataBuffer(ENUM_TaskLogBlockName.TASKLOG_Protect,RTInfo.Task,'write'); % 更新log缓存
      RTInfo.ComStatus = ENUM_ComStatus.ComNormal; % 更新RT信息
      PathModeOut.comStatus = ENUM_ComStatus.ComNormal;
      isComNormal = true;
      printComInfo('[Communication] Normal',1)
    state CommunicationLost
      en:
      RTInfo.Task = ENUM_RTInfo_Task.TaskLog_Protect_Com_Lost;% 更新RTInfo Task
      updateLogDataBuffer(ENUM_TaskLogBlockName.TASKLOG_Protect,RTInfo.Task,'write'); % 更新log缓存
      RTInfo.ComStatus = ENUM_ComStatus.RemoteOrStationLost; % 更新RT信息
      PathModeOut.comStatus = ENUM_ComStatus.RemoteOrStationLost;
      isComNormal = false;
      printComInfo('[Communication] Lost',1)
      if eventEnable_UnexpectedToGoHome
      send(event_goHome_ComLost,FLIGHTMODE.AUTO_TASK)
      end
    (default) -> CommunicationNormal
    CommunicationLost -> CommunicationNormal : [isRemoteConnected&&isStationConnected &&...
        | after(2,sec)]
    CommunicationNormal -> CommunicationLost : [~isRemoteConnected||isStationLostForAWhile]
  state Stall_Protect [parallel]
    settings: executionOrder=21
    state Normal
      en:
    state Stall
      en:
      RTInfo.Task = ENUM_RTInfo_Task.TaskLog_Protect_Stall_Stall;% 更新RTInfo Task
      updateLogDataBuffer(ENUM_TaskLogBlockName.TASKLOG_Protect,RTInfo.Task,'write'); % 更新log缓存
      printComInfo('[Stall] Enter Stall',1)
      RTInfo.StallStatus = ENUM_RTInfo_Stall.StallStatus_InStall; % 更新RT信息
      send(event_stallRecovery,FLIGHTMODE.AUTO_TASK)
      ex:
      RTInfo.Task = ENUM_RTInfo_Task.TaskLog_Protect_Stall_Recovery;% 更新RTInfo Task
      updateLogDataBuffer(ENUM_TaskLogBlockName.TASKLOG_Protect,RTInfo.Task,'write'); % 更新log缓存
      RTInfo.StallStatus = ENUM_RTInfo_Stall.StallStatus_Recovery; % 更新RT信息
      printComInfo('[Stall] Exit Stall',1)
    (default) -> Stall_Protect.Normal : {RTInfo.StallStatus = ENUM_RTInfo_Stall.StallStatus_Normal; }% 更新RT信息
    Stall_Protect.Normal -> Stall : [isStallingForAWhile]
    Stall -> Stall_Protect.Normal : [isGetOutOfStall]
  state BatteryLife_Protect [parallel]
    settings: executionOrder=11
    state BatteryNormal
      en:
      RTInfo.Task = ENUM_RTInfo_Task.TaskLog_Protect_Battery_Normal;% 更新RTInfo Task
      updateLogDataBuffer(ENUM_TaskLogBlockName.TASKLOG_Protect,RTInfo.Task,'write'); % 更新log缓存
      RTInfo.BatteryStatus = ENUM_BatteryStatus.BatteryNormal; % 更新RT信息
      BatteryOut.batteryStatus = ENUM_BatteryStatus.BatteryNormal;
      printComInfo('[BatteryLife] Normal',1)
    state BatteryLow
      en:
      RTInfo.Task = ENUM_RTInfo_Task.TaskLog_Protect_Battery_Low;% 更新RTInfo Task
      updateLogDataBuffer(ENUM_TaskLogBlockName.TASKLOG_Protect,RTInfo.Task,'write'); % 更新log缓存
      RTInfo.BatteryStatus = ENUM_BatteryStatus.BatteryLow; % 更新RT信息
      BatteryOut.batteryStatus = ENUM_BatteryStatus.BatteryLow;
      printComInfo('[BatteryLife] Low',1)
      if eventEnable_UnexpectedToGoHome
      send(event_goHomeThenLand_BatteryLow,FLIGHTMODE.AUTO_TASK)
      end
    state BatterySevereLow
      en:
      RTInfo.Task = ENUM_RTInfo_Task.TaskLog_Protect_Battery_SevereLow;% 更新RTInfo Task
      updateLogDataBuffer(ENUM_TaskLogBlockName.TASKLOG_Protect,RTInfo.Task,'write'); % 更新log缓存
      RTInfo.BatteryStatus = ENUM_BatteryStatus.BatterySevereLow; % 更新RT信息
      BatteryOut.batteryStatus = ENUM_BatteryStatus.BatterySevereLow;
      printComInfo('[BatteryLife] SevereLow',1)
      if eventEnable_UnexpectedToLand
      send(event_land_BatterySevereLow,FLIGHTMODE.AUTO_TASK)
      end
    (default) -> BatteryNormal
    (junction 1508) -> BatteryNormal
    (junction 1506) -> (junction 1508)
    BatteryNormal -> BatteryLow : [isAllBatteryLow]
    BatteryLow -> (junction 1506) [order 2] : [~isAllBatteryLow]
    (junction 1965) -> (junction 1506) [order 2]
    (junction 1965) -> BatteryLow [order 1] : [isAllBatteryLow]
    (junction 1511) -> (junction 1965) : [~isAllBatterySevereLow]
    BatteryLow -> BatterySevereLow [order 1] : [isAllBatterySevereLow && eventEnable_UnexpectedToGoHome]
    BatterySevereLow -> (junction 1511) [order 1]
    BatterySevereLow -> BatterySevereLow [order 2] : [enforceLand]
  state HeightTooLowInHoverUp_Protect [parallel]
    settings: executionOrder=19
    state Normal
      en:
    state HasBeenTooLow
      en:
      RTInfo.Task = ENUM_RTInfo_Task.TaskLog_Protect_HeightInHoverUp_TooLow;% 更新RTInfo Task
      updateLogDataBuffer(ENUM_TaskLogBlockName.TASKLOG_Protect,RTInfo.Task,'write'); % 更新log缓存
      printComInfo('[HeightTooLowInHoverUp_Protect] HasBeenTooLow',1)
      send(event_fix2Rotor2Home2Land,FLIGHTMODE.AUTO_TASK)
      ex:
      RTInfo.Task = ENUM_RTInfo_Task.TaskLog_Protect_HeightInHoverUp_Normal;% 更新RTInfo Task
      updateLogDataBuffer(ENUM_TaskLogBlockName.TASKLOG_Protect,RTInfo.Task,'write'); % 更新log缓存
    (default) -> HeightTooLowInHoverUp_Protect.Normal
    HeightTooLowInHoverUp_Protect.Normal -> HeightTooLowInHoverUp_Protect.HasBeenTooLow : [isHeightLowerThanSwitchHeight_HoverUp]
    HeightTooLowInHoverUp_Protect.HasBeenTooLow -> HeightTooLowInHoverUp_Protect.Normal : [PathModeOut.flightTaskMode == ENUM_FlightTaskMode.GroundStandByMode]
  state HeightTooLowInHoverDown_Protect [parallel]
    settings: executionOrder=10
    state Normal
      en:
      RTInfo.Task = ENUM_RTInfo_Task.TaskLog_Protect_Height_Normal;% 更新RTInfo Task
      updateLogDataBuffer(ENUM_TaskLogBlockName.TASKLOG_Protect,RTInfo.Task,'write'); % 更新log缓存
      RTInfo.FixWingHeightStatus = ENUM_RTInfo_FixHeight.FixWingHeight_Normal; % 更新RT信息
    state HasBeenTooLow
      en:
      RTInfo.Task = ENUM_RTInfo_Task.TaskLog_Protect_Height_TooLow;% 更新RTInfo Task
      updateLogDataBuffer(ENUM_TaskLogBlockName.TASKLOG_Protect,RTInfo.Task,'write'); % 更新log缓存
      RTInfo.FixWingHeightStatus = ENUM_RTInfo_FixHeight.FixWingHeight_TooLow; % 更新RT信息
      printComInfo('[HeightTooLowInFix_Protect] HasBeenTooLow',1)
      % send(event_goHomeThenLand_TooLowInFix,FLIGHTMODE.AUTO_TASK)
    (default) -> HeightTooLowInHoverDown_Protect.Normal
    HeightTooLowInHoverDown_Protect.Normal -> HeightTooLowInHoverDown_Protect.HasBeenTooLow : [isHeightTooLow_HoverDown]
    HeightTooLowInHoverDown_Protect.HasBeenTooLow -> HeightTooLowInHoverDown_Protect.Normal : [PathModeOut.flightTaskMode == ENUM_FlightTaskMode.GroundStandByMode]
  state SensorDegrade_Protect [parallel]
    en,du:
    flag_canContinueFly = canContinueFly;
    flag_isNeedToReturn = isNeedToReturn;
    settings: executionOrder=15
    state Degrade
      en:
      RTInfo.Task = ENUM_RTInfo_Task.TaskLog_Protect_SensorSystem_Degrade;% 更新RTInfo Task
      updateLogDataBuffer(ENUM_TaskLogBlockName.TASKLOG_Protect,RTInfo.Task,'write'); % 更新log缓存
      RTInfo.SensorStatus = ENUM_RTInfo_SensorHealth.SensorRT_Degrade; % 更新RT信息
      if isDebugInfoToShow
      fprintf('\t time %.2f [sec]: SignalIntegrity [Enter Degrade] NeedToReturn!\n',clock_sec);
      end
      if eventEnable_UnexpectedToGoHome
      send(event_goHomeThenLand_SensorDegrade,FLIGHTMODE.AUTO_TASK)
      end
      ex:
      if isDebugInfoToShow
      fprintf('\t time %.2f [sec]: SignalIntegrity [Exit Degrade] NeedToReturn!\n',clock_sec);
      end
    state Normal
      en:
      RTInfo.Task = ENUM_RTInfo_Task.TaskLog_Protect_SensorSystem_Normal;% 更新RTInfo Task
      updateLogDataBuffer(ENUM_TaskLogBlockName.TASKLOG_Protect,RTInfo.Task,'write'); % 更新log缓存
      RTInfo.SensorStatus = ENUM_RTInfo_SensorHealth.SensorRT_Normal; % 更新RT信息
      if isDebugInfoToShow
      fprintf('\t time %.2f [sec]: SignalIntegrity [Enter Normal] Normal!\n',clock_sec);
      end
      du:
    state Fault
      en:
      RTInfo.Task = ENUM_RTInfo_Task.TaskLog_Protect_SensorSystem_Fault;% 更新RTInfo Task
      updateLogDataBuffer(ENUM_TaskLogBlockName.TASKLOG_Protect,RTInfo.Task,'write'); % 更新log缓存
      RTInfo.SensorStatus = ENUM_RTInfo_SensorHealth.SensorRT_Fault; % 更新RT信息
      if isDebugInfoToShow
      fprintf('\t time %.2f [sec]: SignalIntegrity [Enter Fault] canContinueFly!\n',clock_sec);
      end
      send(event_land_SensorNotHealth,FLIGHTMODE.AUTO_TASK)
      ex:
      if isDebugInfoToShow
      fprintf('\t time %.2f [sec]: SignalIntegrity [Exit Fault] canContinueFly!\n',clock_sec);
      end
    (default) -> SensorDegrade_Protect.Normal
    SensorDegrade_Protect.Normal -> (junction 1856)
    (junction 1856) -> Degrade [order 1] : [flag_canContinueFly &&...
        | flag_isNeedToReturn]
    (junction 1856) -> (junction 1886) [order 2]
    Degrade -> (junction 1886)
    (junction 1886) -> Fault : [~flag_canContinueFly]
  state Fense_Protect [parallel]
    en:
    fenseValidDist = TaskParam.fenseDist;
    du:
    updateFenseDist;
    settings: executionOrder=16
    state BeforeUnlock
      en:
      if isDebugInfoToShow
      fprintf('\t time %.2f [sec]: [FENSE] Enter BeforeUnlock!\n',clock_sec);
      end
      RTInfo.FenseStatus = ENUM_RTInfo_Fense.FenseStatus_BeforeUnlock; % 更新RT信息
    state Unlock
      en:
      RTInfo.FenseStatus = ENUM_RTInfo_Fense.FenseStatus_Unlock; % 更新RT信息
      state InFense
        en:
        if isDebugInfoToShow
        fprintf('\t time %.2f [sec]: [FENSE] Enter Unlock, InFense!\n',clock_sec);
        end
        RTInfo.FenseStatus = ENUM_RTInfo_Fense.FenseStatus_In; % 更新RT信息
        du:
        isNotInFense = isOutOfFense(fenseValidDist);
      state OutOfFense
        en:
        RTInfo.Task = ENUM_RTInfo_Task.TaskLog_Protect_Fense_Out;% 更新RTInfo Task
        updateLogDataBuffer(ENUM_TaskLogBlockName.TASKLOG_Protect,RTInfo.Task,'write'); % 更新log缓存
        if isDebugInfoToShow
        fprintf('\t time %.2f [sec]: [FENSE] Enter Unlock, OutOfFense!\n',clock_sec);
        end
        RTInfo.FenseStatus = ENUM_RTInfo_Fense.FenseStatus_Out; % 更新RT信息
        send(event_goHome_NotInFense,FLIGHTMODE.AUTO_TASK)
        du:
        isNotInFense = isOutOfFense(fenseValidDist-0.2e3);
        ex:
        RTInfo.Task = ENUM_RTInfo_Task.TaskLog_Protect_Fense_In;% 更新RTInfo Task
        updateLogDataBuffer(ENUM_TaskLogBlockName.TASKLOG_Protect,RTInfo.Task,'write'); % 更新log缓存
      (default) -> InFense
      OutOfFense -> InFense : [~isNotInFense && after(2,sec)]
      InFense -> OutOfFense : [isNotInFense]
    (default) -> BeforeUnlock
    BeforeUnlock -> Fense_Protect.Unlock : [IN_OnPlane.unlock]
    Fense_Protect.Unlock -> BeforeUnlock : [~IN_OnPlane.unlock]
  state AirspeedFault_Protect [parallel]
    settings: executionOrder=20
    state Work
      state normal
        en:
        printDebugInfo('AirspeedFault_Protect','Enter Normal')
        RTInfo.Task = ENUM_RTInfo_Task.TaskLog_Protect_Airspeed_Normal; % 更新RT信息
        updateLogDataBuffer(ENUM_TaskLogBlockName.TASKLOG_FlightMode,RTInfo.Task,'write'); % 更新log缓存
      state abnormal1
        en:
        printDebugInfo('AirspeedFault_Protect','Enter Abnormal1')
        RTInfo.Task = ENUM_RTInfo_Task.TaskLog_Protect_Airspeed_Fault_1; % 更新RT信息
        updateLogDataBuffer(ENUM_TaskLogBlockName.TASKLOG_FlightMode,RTInfo.Task,'write'); % 更新log缓存
        RTInfo.AttitudeStatus = ENUM_RTInfo_LargeAttitude.LargeAttitude_Abnormal; % 更新RT信息
        if isNeedToRotor
        send(event_fix2Rotor2Home2Land_AirspeedFalut,FLIGHTMODE.AUTO_TASK)
        else
        send(event_goHomeThenLand_AirspeedFalut,FLIGHTMODE.AUTO_TASK)
        end
        du:
        if isNeedToRotor && isUavInFix
        send(event_fix2Rotor2Home2Land_AirspeedFalut,FLIGHTMODE.AUTO_TASK)
        end
      state abnormal2
        en:
        printDebugInfo('AirspeedFault_Protect','Enter Abnormal2')
        RTInfo.Task = ENUM_RTInfo_Task.TaskLog_Protect_Airspeed_Fault_2; % 更新RT信息
        updateLogDataBuffer(ENUM_TaskLogBlockName.TASKLOG_FlightMode,RTInfo.Task,'write'); % 更新log缓存
        RTInfo.AttitudeStatus = ENUM_RTInfo_LargeAttitude.LargeAttitude_Abnormal; % 更新RT信息
        if isNeedToRotor
        send(event_fix2Rotor2Home2Land_AirspeedFalut,FLIGHTMODE.AUTO_TASK)
        else
        send(event_goHomeThenLand_AirspeedFalut,FLIGHTMODE.AUTO_TASK)
        end
        du:
        if isNeedToRotor && isUavInFix
        send(event_fix2Rotor2Home2Land_AirspeedFalut,FLIGHTMODE.AUTO_TASK)
        end
      (default) -> normal
      normal -> abnormal1 : [isNeedToGoHome || ...
          | isNeedToRotor]
          | {PathModeOut.isAirspeedGood = false;
          | PathModeOut.airspeedOffset = TaskParam.airspeedOffset;}
      abnormal1 -> normal [commented out] : [~isLargeAttitudeLong(ComFlightOut.curEuler(2))]
      abnormal1 -> abnormal2 : [isNeedToGoHome && isUavInFix && after(15,sec)]
          | {PathModeOut.isAirspeedGood = false;
          | PathModeOut.airspeedOffset = 1.5*TaskParam.airspeedOffset;}
    (default) -> AirspeedFault_Protect.Work
  state HighWind_Protect [parallel]
    settings: executionOrder=13
    state Normal
      en:
      RTInfo.WindSafeStatus = ENUM_RTInfo_WindSafeStatus.Wind_Normal; % 更新RT信息
    state HasBeenTooLow
      en:
      RTInfo.Task = ENUM_RTInfo_Task.TaskLog_Protect_Wind_VeryHigh;% 更新RTInfo Task
      updateLogDataBuffer(ENUM_TaskLogBlockName.TASKLOG_Protect,RTInfo.Task,'write'); % 更新log缓存
      RTInfo.WindSafeStatus = ENUM_RTInfo_WindSafeStatus.Wind_VeryHigh; % 更新RT信息
      printComInfo('[HighWind_Protect] GoHome by Very High Wind',1)
      if eventEnable_UnexpectedToGoHome
      send(event_goHomeThenLand_VeryHighWind,FLIGHTMODE.AUTO_TASK)
      end
    (default) -> HighWind_Protect.Normal
    HighWind_Protect.Normal -> HighWind_Protect.HasBeenTooLow : [isVeryHighWind] % && isAnyGPSOk]
  state SystemLockInTheAir_Protect [parallel]
    settings: executionOrder=14
    state Normal
    state LockedInTheAir
      en:
      RTInfo.Task = ENUM_RTInfo_Task.Enter_SystemLockInTheAir_Protect_LockedInTheAir; % 更新RT信息
      if isDebugInfoToShow
      fprintf('\t time %.2f [sec]: SystemLockInTheAir_Protect [LockedInTheAir] Enter!\n',clock_sec);
      end
    state UnLockInTheAir
      en:
      RTInfo.Task = ENUM_RTInfo_Task.Enter_SystemLockInTheAir_Protect_UnLockedInTheAir; % 更新RT信息
      if isDebugInfoToShow
      fprintf('\t time %.2f [sec]: SystemLockInTheAir_Protect [UnLockedInTheAir] Enter!\n',clock_sec);
      end
    (default) -> SystemLockInTheAir_Protect.Normal
    SystemLockInTheAir_Protect.Normal -> LockedInTheAir : [0]%[~IN_OnPlane.unlock && isInTheAir]
    LockedInTheAir -> UnLockInTheAir : [IN_OnPlane.unlock && isInTheAir]
    UnLockInTheAir -> LockedInTheAir : [~IN_OnPlane.unlock && isInTheAir]
  data: blockName function_input; message function_input; operation function_input; varargin function_input; flag function_output; flag function_output; validNumOut function_output; flag function_output; out function_output; radarHeight function_input; SampeTime function_input; veld_cmd function_input; y function_output; flag function_output; flag function_output; flag function_output; flag function_output; flag function_output; flag function_output; flag function_output; flag function_output; flag function_output; flag function_output; flag function_output; flag function_output; mode function_input; flag function_output; dist function_output; Rtarget function_input; LL1 function_input; LL2 function_input; flag function_output; flag function_output; heightErr function_input; uavLLA_in function_input; targetLLA_in function_input; headingCmd function_output; flag function_output; posErr function_input; flag function_output; flag function_output; flag function_output; flag function_output; flag function_output; headingCmd function_input; headingNow function_input; dHeading function_output; flag function_output; airspeed_req function_input; groundspeed_req function_input; uavLLA function_input; point1LLA function_input; point2LLA function_input; flag function_output; In_AlgoParams function_input; centerLL function_input; curLL function_input; R function_input; out function_output; flag function_output; flag function_output; flag function_output; value function_input; PathModeOut_out function_output; curLLA_param function_input; startLLA_param function_input; targetLLA_param function_input; PathModeOut_in function_input; mission_item_def_param function_input; uavLLA function_input; point1LLA function_input; point2LLA function_input; dz function_output; flag function_output; flag function_output; flag function_output; flag function_output; flag function_output; flag function_output; enterLLA local; dist_straightForward local; dist_toCenter local; point1LLA function_input; point2LLA function_input; dist_horizontal function_output; flag function_output; flag function_output; flag function_output; flag function_output; posErr function_input; dist function_output; flag function_output; flag function_output; flag function_output; flag function_output; bestpos function_input; flag function_output; out function_output; flag function_output; flag function_output; flag function_output; flag function_output; flag function_output; flag function_output; flag function_output; stableTime0 local; flag function_output; flag function_output; stableTime0 local; headingIN_VerticalMove local; flag function_output; flag function_output; flag function_output; flag function_output; flag function_output; lla function_input; ll0 function_input; p function_output; flag function_output; fenseDist function_input; flag function_output; flag function_output; flag function_output; out function_output; pos function_input; debugInfo function_input; tabspace function_input; varargin function_input; out function_output; pos function_input; lat_deg function_input; modeName function_input; debugInfo function_input; varargin function_input; flag function_output; flag function_output; flag function_output; flag function_output; flag function_output; flag function_output; flag function_output; flag function_output; flag function_output; flag function_output; flag_isNeedToReturn local; flag_canContinueFly local; flag_out function_output; pitch_in function_input; threshold_pitch function_input; flag_out function_output; pitch_in function_input; threshold_pitch function_input; flag_out function_output; Vd_in function_input; flag function_output; flag function_output; flag function_output; flag function_output; flag_out function_output; current_in function_input; threshold_current function_input; flag_out function_output; current_in function_input; threshold_current function_input; flag function_output; flag function_output; flag function_output; flag function_output; flag function_output; flag function_output; clock_sec input; Ts input; IN_MAV input Bus: BUS_MAVLINK_TO_FIRM; TASK_NAVIMode output Enum: TASK_NAVIModeType; IN_NAVI input Bus: BUS_NAVI_TO_FIRM; IN_SignalIntegrity input Bus: BUS_NAVI_SensorSignalIntegrity; IN_OnPlane input Bus: BUS_ONPLANE_FEEDBACK; IN_SENSOR input Bus: BUS_SENSOR; PathModeOut output Bus: BUS_TASK_PATH_OutParam; ComFlightOut output Bus: BUS_TASK_COMMON_OutParam size=1; targetLLA local; tempIdx local; temp_AlgoParams local Bus: BUS_TASK_PATH_AlgoParam; arriveFlag local; startLLA local; DebugParam local Bus: BUS_TASK_DEBUG_STEP; this_mission_item_def local Bus: mavlink_mission_item_def; nextMode local; isContinuePath local; idxStartPathPoint local; headingMode local; PayloadControlOut output Bus: BUS_TASK_PAYLOAD size=1; doHeightCmdKeepAfterHeightSwitch local; CmdParam_altitude local; CmdParam_cameraTrigDist local; BatteryOut output Bus: BUS_TASK_BATTERY size=1; TaskModeBeforeAirStandBy local; HeightCmdBeforeAirStandBy local; isComNormal local boolean; isAttitudeStable_globalvar local; isAutoMode_globalvar local boolean; RTInfo output Bus: BUS_TASK_RTInfo; hasTaskStarted_globalbar local; HeadingCmdBeforeAirStandBy local; preTaskMode local Enum: ENUM_FlightTaskMode; isNotInFense local; typeAutoModePre local; HomeParam output Bus: BUS_TASK_HomeParam size=1; OUT_ONPLANESTORE output Bus: BUS_ONPLANE_STORE size=1; isArrive1stPointInPathMode local; idxTransitPoint local; landPosMode local Enum: ENUM_LandMode; WindParamOut output Bus: Bus_TASK_WindParam; isLatLonOK_Land local; hasTakeOff local; resetPathProgram local; fenseValidDist local; FlightPerfParam data_store_memory; IN_FlightPerf input; IN_WindNED input; resetRTlog local; logDataOut output Bus: BUS_TASK_SingleLog size=TASK_PARAM_V1000.logDataOutSize; logDataBuffer output Bus: BUS_TASK_SingleLog size=TASK_PARAM_V1000.logDataBufferSize; enterNum_Land local; TaskParam data_store_memory; isDebugInfoToShow data_store_memory; isAirspeedGood local =true; LLA_EnterTakeOffMode local size=[1,3] =[0,0,0]
  events: event_goFirstPoint local FUNCTION_CALL_EVENT; event_goHomePoint local FUNCTION_CALL_EVENT; event_arrivePoint local FUNCTION_CALL_EVENT; event_goLastPoint local FUNCTION_CALL_EVENT; event_getNearHome local FUNCTION_CALL_EVENT; manual_goHomePoint local FUNCTION_CALL_EVENT; manual_goIntoPath local FUNCTION_CALL_EVENT; manual_takeOff local FUNCTION_CALL_EVENT; manual_airStandBy local FUNCTION_CALL_EVENT; manual_hoverAdjust local FUNCTION_CALL_EVENT; manual_rotor2Fix local FUNCTION_CALL_EVENT; manual_hoverUp local FUNCTION_CALL_EVENT; manual_fix2Rotor local FUNCTION_CALL_EVENT; manual_switchHeight local FUNCTION_CALL_EVENT; auto_gotoNextMode local FUNCTION_CALL_EVENT; manual_groundStandBy local FUNCTION_CALL_EVENT; event_goMidPoint local FUNCTION_CALL_EVENT; manual_continueProfile local FUNCTION_CALL_EVENT; event_finishPath local FUNCTION_CALL_EVENT; manual_hoverDown local FUNCTION_CALL_EVENT; payload_beginWork local FUNCTION_CALL_EVENT; payload_stopWork local FUNCTION_CALL_EVENT; manual_land local FUNCTION_CALL_EVENT; auto_goto_HoverAdjustMode local FUNCTION_CALL_EVENT; event_land_SensorNotHealth local FUNCTION_CALL_EVENT; event_goHome_NotInFense local FUNCTION_CALL_EVENT; manual_rotorGoUp local FUNCTION_CALL_EVENT; event_goHomeThenLand_BatteryLow local FUNCTION_CALL_EVENT; event_land_BatterySevereLow local FUNCTION_CALL_EVENT; event_goHome_ComLost local FUNCTION_CALL_EVENT; event_stallRecovery local FUNCTION_CALL_EVENT; event_goHomeThenLand_StallRecovery local FUNCTION_CALL_EVENT; event_startTaskFromAir local FUNCTION_CALL_EVENT; event_oneKeyGoHome local FUNCTION_CALL_EVENT; event_land_GScommand local FUNCTION_CALL_EVENT; event_gotoWaitForContinue local FUNCTION_CALL_EVENT; event_goHomeThenLand_TooLowInFix local FUNCTION_CALL_EVENT; event_directToHoverFromGoHome local FUNCTION_CALL_EVENT; event_goHomeThenLand_VeryHighWind local FUNCTION_CALL_EVENT; event_goHomeThenLand_SensorDegrade local FUNCTION_CALL_EVENT; event_homeChanged local FUNCTION_CALL_EVENT; event_fix2Rotor2Home2Land local FUNCTION_CALL_EVENT; event_verticalMove local FUNCTION_CALL_EVENT; event_goHomeThenLand_AirspeedFalut local FUNCTION_CALL_EVENT; event_single_groundMode local FUNCTION_CALL_EVENT; event_single_hoverAdjustMode local FUNCTION_CALL_EVENT; event_single_takeOffMode local FUNCTION_CALL_EVENT; event_single_rotor2FixMode local FUNCTION_CALL_EVENT; event_single_hoverUpMode local FUNCTION_CALL_EVENT; event_single_hoverDownMode local FUNCTION_CALL_EVENT; event_single_fix2RotorMode local FUNCTION_CALL_EVENT; event_single_landMode local FUNCTION_CALL_EVENT; event_single_pathMode local FUNCTION_CALL_EVENT; event_single_airStandByMode local FUNCTION_CALL_EVENT; event_single_stallRecoveryMode local FUNCTION_CALL_EVENT; event_single_goHomeMode local FUNCTION_CALL_EVENT; event_goHomeThenLand_LargeOffsetInLand local FUNCTION_CALL_EVENT; event local FUNCTION_CALL_EVENT; event1 local FUNCTION_CALL_EVENT; event_fix2Rotor2Home2Land_AirspeedFalut local FUNCTION_CALL_EVENT
  function updateLogDataBuffer(blockName,message,operation,varargin):
    | function updateLogDataBuffer(blockName,message,operation,varargin)
    | persistent pIdx pBufferIdx preTime
    | if isempty(pIdx)
    |     pIdx = 0;
    |     pBufferIdx = 0;
    |     preTime = clock_sec;
    | end
    | %%
    | if nargin == 4
    |     var_input = varargin{1};
    | else
    |     var_input = zeros(5,1);
    | end
    | bufferIdx = pBufferIdx;
    | idx = pIdx;
    | thisTime = clock_sec;
    | switch operation
    |     case 'write'
    |         thisTime = clock_sec;
    |         if preTime ~= thisTime
    |             idx = 0; % 同一时间刻度下, 不同信息的先后顺序
    |         end
    |         if bufferIdx < length(logDataBuffer)
    |             bufferIdx = bufferIdx + 1;
    |             idx = idx + 1;
    |             temp = formatLogStruct(blockName,message,var_input);
    |             tempData.time_sec = clock_sec;
    |             tempData.idx = idx;
    |             tempData.blockName = blockName;
    |             tempData.message = message;
    |             tempData.var1 = temp.var1;
    |             logDataBuffer(bufferIdx) = tempData;
    |         end
    |     case 'read'
    |         for i_out = 1:1 %AlgoParams.logDataOutSize
    |             %             logDataOut(i_out) = resetLogStruct; % 置零
    |             logDataOut(i_out).time_sec = 0;
    |             logDataOut(i_out).idx = 0;
    |             logDataOut(i_out).blockName = ENUM_TaskLogBlockName(0);
    |             logDataOut(i_out).message = ENUM_RTInfo_Task(0);
    |             logDataOut(i_out).var1 = zeros(5,1);
    |             if bufferIdx > 0
    |                 logDataOut(i_out) = logDataBuffer(bufferIdx);
    |                 %                 logDataBuffer(bufferIdx) = resetLogStruct;
    |                 logDataBuffer(bufferIdx).time_sec = 0;
    |                 logDataBuffer(bufferIdx).idx = 0;
    |                 logDataBuffer(bufferIdx).blockName = ENUM_TaskLogBlockName(0);
    |                 logDataBuffer(bufferIdx).message = ENUM_RTInfo_Task(0);
    |                 logDataBuffer(bufferIdx).var1 = zeros(5,1);
    |                 bufferIdx = bufferIdx - 1;
    |             end
    |         end
    | end
    | preTime = thisTime;
    | pBufferIdx = bufferIdx;
    | pIdx = idx;
    | %% 子函数
    | function log = resetLogStruct
    | log.time_sec = 0;
    | log.idx = 0;
    | log.blockName = ENUM_TaskLogBlockName(0);
    | log.message = ENUM_RTInfo_Task(0);
    | log.var1 = zeros(5,1);
    | 
    | function log = formatLogStruct(blockName,message,var_input)
    | log.message = message;
    | log.var1 = zeros(5,1);
    | switch blockName
    |     case ENUM_TaskLogBlockName.TASKLOG_FlightMode
    |         log.var1(1) = ComFlightOut.curLLA(1);
    |         log.var1(2) = ComFlightOut.curLLA(2);
    |         log.var1(3) = ComFlightOut.curLLA(3);
    |         log.var1(4) = norm(ComFlightOut.curAirSpeed);
    | %         log.var1(5) = PathModeOut.uavMode;
    |         switch message             
    |             case {ENUM_RTInfo_Task.HoverUp_INIT_ContinueHoverUpDown,...
    |                     ENUM_RTInfo_Task.Enter_AutoMode_AirStandBy_Doing,...
    |                     ENUM_RTInfo_Task.Enter_AutoMode_HoverDown_HeightDown,...
    |                     ENUM_RTInfo_Task.Enter_AutoMode_HoverUp_Doing,...
    |                     ENUM_RTInfo_Task.Enter_AutoMode_HoverUp_LevelAttitude}
    |                 log.var1 = zeros(5,1);
    |                 log.var1(1) = PathModeOut.turnCenterLL(1);
    |                 log.var1(2) = PathModeOut.turnCenterLL(2);  
    |                 log.var1(3) = ComFlightOut.curLLA(3);
    | %             case {ENUM_RTInfo_Task.Fix2Rotor_ToGo_Complete_Con1,...
    | %                     ENUM_RTInfo_Task.Fix2Rotor_ToGo_Complete_Con2}
    | %                 log.var1(1) = ComFlightOut.curLLA(1);
    | %                 log.var1(2) = ComFlightOut.curLLA(2);
    | %                 log.var1(3) = ComFlightOut.curLLA(3);
    | %                 log.var1(4) = norm(ComFlightOut.curAirSpeed);
    | %                 log.var1(5) = PathModeOut.uavMode;                
    |         end
    |     otherwise
    |         switch message
    |             case {ENUM_RTInfo_Task.VerticalMove_BeforeGoHome_Enter_No,ENUM_RTInfo_Task.VerticalMove_BeforeGoHome_Enter_Yes,...
    |                     ENUM_RTInfo_Task.VerticalMove_BeforePath_Enter_No,ENUM_RTInfo_Task.VerticalMove_BeforePath_Enter_Yes}
    |                 log.var1 = var_input;
    |                 log.var1(1) = var_input(1);
    |                 log.var1(2) = var_input(2);
    |                 log.var1(3) = var_input(3);
    |                 log.var1(4) = var_input(4);
    |                 log.var1(5) = var_input(5);
    |             case ENUM_RTInfo_Task.TaskLog_Payload_Camera_Shot
    |                 log.var1 = [PayloadControlOut.CAMERA.trigger;
    |                     PayloadControlOut.CAMERA.LLA(1);
    |                     PayloadControlOut.CAMERA.LLA(2);
    |                     PayloadControlOut.CAMERA.LLA(3);
    |                     0;];
    |             case ENUM_RTInfo_Task.TaskLog_Mav_CmdChange
    |                 log.var1(1) = IN_MAV.mavlink_msg_id_command_long.command;
    |                 log.var1(2) = IN_MAV.mavlink_msg_id_command_long.param1;
    |             case ENUM_RTInfo_Task.TaskLog_Protect_Height_TooLow
    |                 log.var1(1) = ComFlightOut.curLLA(3);
    |             case ENUM_RTInfo_Task.TaskLog_Protect_Stall_Stall
    |                 log.var1(1) = norm(ComFlightOut.curAirSpeed);
    |                 log.var1(2) = norm(ComFlightOut.curGroundSpeed);
    |                 log.var1(3) = ComFlightOut.curLLA(3);
    |             case {ENUM_RTInfo_Task.TaskLog_Protect_Battery_Low,ENUM_RTInfo_Task.TaskLog_Protect_Battery_SevereLow}
    |                 log.var1(1) = IN_MAV.mavlink_msg_mission_current(1).remaining;
    |                 log.var1(2) = IN_FlightPerf.flagGoHomeNow;
    |             case ENUM_RTInfo_Task.TaskLog_Protect_Wind_VeryHigh
    |                 log.var1(1) = IN_WindNED.windSpeed_ms;
    |                 log.var1(2) = IN_WindNED.windHeading_rad;
    |             case {ENUM_RTInfo_Task.TaskLog_Input_HomeChange_GS,...
    |                     ENUM_RTInfo_Task.TaskLog_Input_HomeChange_KeyBoard,...
    |                     ENUM_RTInfo_Task.TaskLog_Input_HomeChange_Path,...
    |                     ENUM_RTInfo_Task.TaskLog_Input_HomeChange_TakeOff}
    |                 log.var1(1) = ComFlightOut.curHomeLLA(1);
    |                 log.var1(2) = ComFlightOut.curHomeLLA(2);
    |                 log.var1(3) = ComFlightOut.curHomeLLA(3);
    |             case {ENUM_RTInfo_Task.TaskLog_Protect_HeightInHoverUp_TooLow,...
    |                     ENUM_RTInfo_Task.TaskLog_Protect_HeightInHoverUp_Normal}
    |                 log.var1(1) = ComFlightOut.curLLA(3);
    |                 log.var1(2) = CmdParam_altitude;
    |                 log.var1(3) = ComFlightOut.curAirSpeed;
    |                 log.var1(4) = ComFlightOut.curGroundSpeed;
    |         end
    | end
    | log.var1(5) = double(IN_MAV.mavlink_msg_mission_current(1).remaining)/100;
    | if sum(var_input) ~= 0
    |     log.var1 = var_input; % 输入的优先级高
    | end
  function flag = isUavInRotor2Fix:
    | function flag = isUavInRotor2Fix
    | flag = false;
    | if PathModeOut.uavMode == ENUM_UAVMode.Rotor2Fix
    |     flag = true;
    | end
  function flag = isStationLostForAWhile:
    | function flag = isStationLostForAWhile
    | persistent lastNotLostTime lostTime0
    | if isempty(lastNotLostTime)
    |     lastNotLostTime = 0;
    |     lostTime0 = 0;
    | end
    | if isStationConnected
    |     lastNotLostTime = clock_sec; 
    | else
    |     lostTime0 = clock_sec;
    | end
    | flag = false;
    | if lostTime0 - lastNotLostTime > Ts %IN_OnPlane.stationLostTimeSec 输入通断信号已经是累计失联时间后的标志
    |     flag = true;
    | end
  function du_func:
    | function du_func
    | persistent preFlightControlMode
    | if isempty(preFlightControlMode)
    |     preFlightControlMode = PathModeOut.flightControlMode;
    | end
    | if preFlightControlMode ~= PathModeOut.flightControlMode
    |     printDebugInfo('ALL','flightControlMode Changde!')
    |     RTInfo.Task = ENUM_RTInfo_Task.FlightControlMode_Changde; % 更新RT信息
    |     updateLogDataBuffer(ENUM_TaskLogBlockName.TASKLOG_FlightMode,RTInfo.Task,'write',[double(preFlightControlMode);double(PathModeOut.flightControlMode);0;0;0]); % 更新log缓存
    | end
    | preFlightControlMode = PathModeOut.flightControlMode;
    | %
    | updateLogDataBuffer(ENUM_TaskLogBlockName.TASKLOG_None,ENUM_RTInfo_Task(0),'read')
  function updateInput:
    | function updateInput
    | %% ComFlightOut结构体中HomeLLA相关量的计算逻辑比较复杂
    | persistent pre_mission_item_def0 isValid_mavlink_msg_groundHomeLLA taskMode_lastTick hasTakeOff
    | if isempty(pre_mission_item_def0)
    |     hasTakeOff = false;
    |     isValid_mavlink_msg_groundHomeLLA = false;
    |     pre_mission_item_def0 = [IN_MAV.mavlink_mission_item_def(1).x,IN_MAV.mavlink_mission_item_def(1).y, IN_MAV.mavlink_mission_item_def(1).z];
    |     taskMode_lastTick = ENUM_FlightTaskMode.GroundStandByMode;
    |     ComFlightOut.curHomeLLA = [0 0 0];
    |     ComFlightOut.groundHomeLLA = [0 0 0];
    | end
    | if PathModeOut.flightTaskMode == ENUM_FlightTaskMode.TakeOffMode
    |     hasTakeOff = true;
    | end
    | %% 处理home点更新
    | if ~isValid_mavlink_msg_groundHomeLLA && ...
    |         (IN_MAV.mavlink_msg_groundHomeLLA(1) ~= 0 && IN_MAV.mavlink_msg_groundHomeLLA(2) ~= 0)
    |     % 收到mavlink_msg_groundHomeLLA有效值，更新homeLLA
    |     ComFlightOut.curHomeLLA = IN_MAV.mavlink_msg_groundHomeLLA;
    |     isValid_mavlink_msg_groundHomeLLA = true; % 管家获取到有效的home点位置
    |     RTInfo.Task = ENUM_RTInfo_Task.TaskLog_Input_HomeChange_GS;% 更新RTInfo Task
    |     updateLogDataBuffer(ENUM_TaskLogBlockName.TASKLOG_ParserInput,RTInfo.Task,'write'); % 更新log缓存
    | end
    | cur_mission_item_def0 = [IN_MAV.mavlink_mission_item_def(1).x,IN_MAV.mavlink_mission_item_def(1).y, IN_MAV.mavlink_mission_item_def(1).z];
    | if isValid_mavlink_msg_groundHomeLLA
    |     if ~isequal(pre_mission_item_def0,cur_mission_item_def0)
    |         % 当重置home点后,【mission_item_def(1).x,mission_item_def(1).y, mission_item_def(1).z】改变，进行一次homeLLA更新
    |         pre_mission_item_def0 = cur_mission_item_def0;
    |         curHomePoint = reshape(double(cur_mission_item_def0),1,[]);
    |         curHomePoint0 = IN_MAV.mavlink_msg_groundHomeLLA;
    |         tempLLA = updateHomePoint(curHomePoint,curHomePoint0);
    |         ComFlightOut.curHomeLLA(1) = tempLLA(1);
    |         ComFlightOut.curHomeLLA(2) = tempLLA(2);
    |         if 0 % 暂时屏蔽
    |             send(event_homeChanged,FLIGHTMODE.AUTO_TASK.MODE_HOVERADJUST);
    |         end
    |         RTInfo.Task = ENUM_RTInfo_Task.TaskLog_Input_HomeChange_Path;% 更新RTInfo Task
    |         updateLogDataBuffer(ENUM_TaskLogBlockName.TASKLOG_ParserInput,RTInfo.Task,'write'); % 更新log缓存
    |     else
    |         % 当由地面模式变为TakeOff模式时，将起飞点位置更新为Home点位置
    |         enableHomeUpdate_whileTakeOff = true;
    |         if enableHomeUpdate_whileTakeOff
    |             if taskMode_lastTick == ENUM_FlightTaskMode.GroundStandByMode && ...
    |                     PathModeOut.flightTaskMode == ENUM_FlightTaskMode.TakeOffMode % 进入TakeOff模式
    |                 LLA_EnterTakeOffMode = reshape(double(IN_NAVI.lla),1,[]); % 进入TakeOff模式时刻的LLA
    |                 dpos = [111e3*(ComFlightOut.curHomeLLA(1)-LLA_EnterTakeOffMode(1)),...
    |                     111e3*(ComFlightOut.curHomeLLA(2)-LLA_EnterTakeOffMode(2)),...
    |                     ComFlightOut.curHomeLLA(3)-LLA_EnterTakeOffMode(3)];
    |                 fprintf('Enter TakeOff mode, update Home:\n\t%.7f->%.7f,%.2fm\n\t%.7f->%.7f,%.2fm\n\t%.2f->%.2f,%.2fm\n',...
    |                     ComFlightOut.curHomeLLA(1),LLA_EnterTakeOffMode(1),dpos(1),...
    |                     ComFlightOut.curHomeLLA(2),LLA_EnterTakeOffMode(2),dpos(2),...
    |                     ComFlightOut.curHomeLLA(3),LLA_EnterTakeOffMode(3),dpos(3));
    |                 ComFlightOut.curHomeLLA = LLA_EnterTakeOffMode;
    |                 ComFlightOut.groundHomeLLA = ComFlightOut.curHomeLLA;
    |                 RTInfo.Task = ENUM_RTInfo_Task.TaskLog_Input_HomeChange_TakeOff;% 更新RTInfo Task
    |                 updateLogDataBuffer(ENUM_TaskLogBlockName.TASKLOG_ParserInput,RTInfo.Task,'write'); % 更新log缓存
    |             end
    |         end
    |     end
    | end
    | %% Home点变动与否
    | PathModeOut.isHomeChangedAfterTakeOff = false;
    | if norm(LLA_EnterTakeOffMode) ~= 0 
    |     % LLA_EnterTakeOffMode赋值完成后，即起飞后
    |     homeOffset = distOfTwoLL(LLA_EnterTakeOffMode(1:2),ComFlightOut.curHomeLLA(1:2));
    |     if homeOffset < 20 % 判断home点在起飞后没有变很远
    |         PathModeOut.isHomeChangedAfterTakeOff = false;
    |     else
    |         PathModeOut.isHomeChangedAfterTakeOff = true;
    |     end
    | end
    | %% 
    | if PathModeOut.flightTaskMode == ENUM_FlightTaskMode.GroundStandByMode && ~hasTakeOff
    |     ComFlightOut.groundHomeLLA = ComFlightOut.curHomeLLA;
    | end
    | taskMode_lastTick = PathModeOut.flightTaskMode;
    | %%
    | ComFlightOut.curVelNED = reshape(double(IN_NAVI.velNED),1,[]);
    | ComFlightOut.curSpeed = reshape(double(norm(IN_NAVI.velNED(1:2))),1,[]);
    | 
    | if IN_SignalIntegrity.SensorStatus.airspeed1 ~= ENUM_SensorHealthStatus.Health % double(IN_SENSOR.airspeed1.airspeed) == 0 ||
    |     ComFlightOut.curAirSpeed = reshape(double(norm(IN_NAVI.velNED(1:2))),1,[]);
    | else
    |     ComFlightOut.curAirSpeed = double(IN_SENSOR.airspeed1.airspeed_indicate); % 指示空速
    | end
    | if ~PathModeOut.isAirspeedGood
    |     ComFlightOut.curAirSpeed = reshape(double(norm(IN_NAVI.velNED(1:2))),1,[]) - PathModeOut.airspeedOffset; %;
    | end
    | 
    | ComFlightOut.curEuler = reshape(double(IN_NAVI.eulerd_yaw_pitch_roll*pi/180),1,[]);
    | ComFlightOut.curWB = reshape(double(IN_NAVI.gyro_correct),1,[]);
    | ComFlightOut.curPosNED = reshape(double(IN_NAVI.posNED),1,[]);
    | ComFlightOut.curLLA = reshape(double(IN_NAVI.lla),1,[]);
    | ComFlightOut.curGroundSpeed = reshape(double(norm(IN_NAVI.velNED(1:3))),1,[]);
    | ComFlightOut.curAccZ = double(calAccZ);
    | ComFlightOut.curWindSpeed = 0;
    | ComFlightOut.curAlpha = 0;
    | ComFlightOut.curBeta = 0;
    | ComFlightOut.velocityElevation = 0;
    | ComFlightOut.velocityDeclination = 0;
    | % if mavlink_msg_groundHomeLLA(1) == 0 % 若从地面站接收的home点无效,则使用组合导航获取的初始点作为home，只用其高度
    | %     ComFlightOut.groundHomeLLA = IN_NAVI.refloc.';
    | % else
    | %     ComFlightOut.groundHomeLLA = mavlink_msg_groundHomeLLA;
    | % end
    | % 计算风速
    | ComFlightOut.curWindSpeed = double(IN_SENSOR.airspeed1.airspeed_true) - ComFlightOut.curGroundSpeed; % 正表示风从机头方向来
    | % 计算风角
    | if ComFlightOut.curAirSpeed> 2
    |     ComFlightOut.velocityElevation = atan(-ComFlightOut.curVelNED(3)/ComFlightOut.curAirSpeed);
    | else
    |     ComFlightOut.velocityElevation = ComFlightOut.curEuler(2);
    | end
    | if norm(ComFlightOut.curVelNED(1:2)) > 2
    |     ComFlightOut.velocityDeclination = atan2(ComFlightOut.curVelNED(2),ComFlightOut.curVelNED(1));
    | else
    |     ComFlightOut.velocityDeclination = ComFlightOut.curEuler(1);
    | end
    | ComFlightOut.curAlpha = ComFlightOut.curEuler(2) - ComFlightOut.velocityElevation;
    | ComFlightOut.curBeta = angdiff(ComFlightOut.curEuler(1),ComFlightOut.velocityDeclination);
    | % 计算相对home点的高度
    | temp = ComFlightOut.curLLA(3);
    | ComFlightOut.curLLA(3) = temp - ComFlightOut.groundHomeLLA(3); % 海拔高转换为高度
    | ComFlightOut.curHeightForControl = temp - ComFlightOut.groundHomeLLA(3); % 海拔高转换为高度
    | % 雷达高处理
    | radarHeight = double(IN_SENSOR.radar1.Range);
    | if PathModeOut.flightTaskMode == ENUM_FlightTaskMode.LandMode
    |     radarHeight = radarHeightCorrect(radarHeight, Ts, PathModeOut.maxClimbSpeed);
    | end
    | % 起飞降落相对高度
    | if IN_SignalIntegrity.SensorStatus.radar1 == ENUM_SensorHealthStatus.Health && ... % 处于起飞或着陆模式时
    |         radarHeight ~= 0 && radarHeight < TaskParam.minHeightInFix && ...
    |         PathModeOut.uavMode ~= ENUM_UAVMode.Fix
    |     switch PathModeOut.flightTaskMode
    |         case ENUM_FlightTaskMode.LandMode % 着陆时，用于控制的高度curHeightForControl使用GPS融合高
    |             if ~isHomeChangeAfterTakeOff % 降落阶段，如果没改过Home点，则进行高度校验，满足条件则使用radar高参考
    |                 if abs(double(IN_NAVI.lla(3))-ComFlightOut.groundHomeLLA(3)-radarHeight) < 15
    |                     ComFlightOut.curLLA(3) = radarHeight;
    |                 end
    |             else % 降落阶段，如果改过Home点，则不进行高度校验，使用radar高参考，此时不假设更改home后高度不变，因此无法进行高度校验
    |                 ComFlightOut.curLLA(3) = radarHeight;
    |             end
    |         case {ENUM_FlightTaskMode.TakeOffMode, ENUM_FlightTaskMode.GroundStandByMode}
    |             ComFlightOut.curLLA(3) = radarHeight;
    |             ComFlightOut.curHeightForControl = double(radarHeight);
    |         case ENUM_FlightTaskMode.HoverAdjustMode
    |             if preTaskMode == ENUM_FlightTaskMode.TakeOffMode % 前置为起飞模式
    |                 ComFlightOut.curLLA(3) = radarHeight;
    |                 ComFlightOut.curHeightForControl = double(radarHeight);
    |             end
    |             if preTaskMode == ENUM_FlightTaskMode.LandMode % 前置为着陆模式
    |                 ComFlightOut.curLLA(3) = radarHeight;
    |             end
    |         case ENUM_FlightTaskMode.GoHomeMode
    |             % 存在一些隐患
    |     end
    | end
    | % 相对高度为正
    | ComFlightOut.curLLA(3) = abs(ComFlightOut.curLLA(3));
    | % gps时效后对水平速度置零
    | if 0 && ~isAnyGPSOk
    |     ComFlightOut.curVelNED(1) = 0;
    |     ComFlightOut.curVelNED(2) = 0;
    | end
    | %% 子函数
    | function out = updateHomePoint(curHomePoint,curHomePoint0)
    | persistent preHomePoint
    | if isempty(preHomePoint)
    |     preHomePoint = curHomePoint0;
    | end
    | if norm(preHomePoint(1:2)-curHomePoint(1:2)) > 5/111e3 && ...
    |         curHomePoint(1) ~= 0 && curHomePoint(2) ~= 0
    |     preHomePoint = curHomePoint;
    | end
    | out = preHomePoint;
  function validNumOut = calValidPointNum:
    | function validNumOut = calValidPointNum
    | persistent isComplete validPathNum
    | if isempty(isComplete)
    |     isComplete = false;
    |     validPathNum = 0;
    | end
    | maxNum = TaskParam.maxPathPointNum;
    | nanFlag = TaskParam.nanFlag;
    | if isDataRefresh(IN_MAV.mavlink_mission_item_def,maxNum,nanFlag) % 检测航点是否更新
    |     isComplete = false;
    | end
    | % 计算有效航点数
    | if ~isComplete && ...
    |         PathModeOut.flightTaskMode == ENUM_FlightTaskMode.GroundStandByMode % 仅在地面模式时计算
    |     validNum = 0;
    |     homeLL = ComFlightOut.curHomeLLA(1:2);
    |     for i = 1:maxNum
    |         if IN_MAV.mavlink_mission_item_def(i).x == nanFlag || (IN_MAV.mavlink_mission_item_def(i).x == 0 && IN_MAV.mavlink_mission_item_def(i).y == 0) % 0只是暂时的
    |             validNum = i-1;
    |             break;
    |         else
    |             validNum = i;
    |             tmpPathLL = [IN_MAV.mavlink_mission_item_def(i).x,IN_MAV.mavlink_mission_item_def(i).y];
    |             tmpDist = distOfTwoLL(tmpPathLL,homeLL);
    |             if tmpDist > RTInfo.maxDist_Path2Home
    |                 RTInfo.maxDist_Path2Home = tmpDist;
    |             end
    |         end
    |     end
    | %     if i == maxNum
    | %         validNum = maxNum;
    | %     end
    |     if validNum > 1
    |         isComplete = true;
    |         validPathNum = validNum;
    |     end
    | end
    | 
    | validNumOut = validPathNum;
    | %% 子函数
    | function flag = isDataRefresh(pathdata,maxNum,nanFlag)
    | persistent preSum
    | if isempty(preSum)
    |     preSum = 0;
    | end
    | flag = false;
    | sum = 0;
    | for i = 2:maxNum % 从第2个数据点开始，不考虑home点
    |     if pathdata(i).x ~= nanFlag
    |         sum = sum + double(i*pathdata(i).x + 1.1*i*pathdata(i).y);
    |     end
    | end
    | if preSum ~= sum
    |     flag = true;
    | end
    | preSum = sum;
  function flag = isAttitudeStable:
    | function flag = isAttitudeStable
    | persistent rollset pitchset
    | if isempty(rollset)
    |     num = min(ceil(1/Ts),100); % 
    |     rollset = -999*ones(num,1);
    |     pitchset = -999*ones(num,1);
    | end
    | flag = false;
    | rollset(2:end) = rollset(1:end-1);
    | pitchset(2:end) = pitchset(1:end-1);
    | 
    | rollset(1) = ComFlightOut.curEuler(3);
    | pitchset(1) = ComFlightOut.curEuler(2);
    | 
    | if max(abs(rollset(:))) <= TaskParam.threshold_deg_attiStable*pi/180 && ...
    |         max(abs(pitchset(:))) <= (10+TaskParam.threshold_deg_attiStable)*pi/180
    |     flag = true;
    | end
  function updatePreAndCurPathPoint:
    | function updatePreAndCurPathPoint
    | if PathModeOut.prePointNum == 0 || PathModeOut.currentPointNum == 0
    |     return;
    | end
    | % 前置航点
    | tempIdx = PathModeOut.prePointNum;
    | PathModeOut.prePathPoint_LLA = double([IN_MAV.mavlink_mission_item_def(tempIdx).x,...
    |     IN_MAV.mavlink_mission_item_def(tempIdx).y, IN_MAV.mavlink_mission_item_def(tempIdx).z]);
    | % 当前目标航点
    | tempIdx = PathModeOut.currentPointNum;
    | PathModeOut.curPathPoint_LLA = double([IN_MAV.mavlink_mission_item_def(tempIdx).x,...
    |     IN_MAV.mavlink_mission_item_def(tempIdx).y, IN_MAV.mavlink_mission_item_def(tempIdx).z]);
  function out = calAccZ:
    | function out = calAccZ
    | if IN_SignalIntegrity.SensorSelect.IMU == 1
    |     out = IN_SENSOR.IMU1.accel_z;
    | elseif IN_SignalIntegrity.SensorSelect.IMU == 2
    |     out = IN_SENSOR.IMU2.accel_z;
    | elseif IN_SignalIntegrity.SensorSelect.IMU == 3
    |     out = IN_SENSOR.IMU3.accel_z;
    | elseif IN_SignalIntegrity.SensorSelect.IMU == 0
    |     out = 1/3*(IN_SENSOR.IMU1.accel_z+IN_SENSOR.IMU2.accel_z+IN_SENSOR.IMU3.accel_z);
    | else
    |     out = IN_SENSOR.IMU1.accel_z;
    | end
  function updatePathModeOut:
    | function updatePathModeOut
    | % 更新输入
    | PathModeOut.turnRadiusCmd = TaskParam.turnR;
    | if PathModeOut.flightTaskMode == ENUM_FlightTaskMode.PathFollowMode || ...
    |         PathModeOut.flightTaskMode == ENUM_FlightTaskMode.GoHomeMode
    |     PathModeOut.airspeedCmd = max(TaskParam.minAirspeed_fixAllowed,IN_FlightPerf.economicAirspeed);
    |     PathModeOut.airspeedCmd = min(PathModeOut.airspeedCmd,30);
    | else
    |     PathModeOut.airspeedCmd = TaskParam.minAirspeed_fixAllowed;
    | end
    | PathModeOut.switchHeight = CmdParam_altitude;
    | PathModeOut.isHeadingRotate_OnGround = IN_NAVI.isHeadingRotateFlag && PathModeOut.flightTaskMode == ENUM_FlightTaskMode.GroundStandByMode;
  function y = radarHeightCorrect(radarHeight, SampeTime, veld_cmd):
    | function y = radarHeightCorrect(radarHeight, SampeTime, veld_cmd)
    | persistent heightSmooth preHeight
    | curHeight = double(radarHeight);
    | if isempty(heightSmooth)
    |     preHeight = curHeight;
    |     heightSmooth = curHeight;
    | end
    | maxHeightVel = 1.5*veld_cmd;
    | curHeight_correct = curHeight;
    | if heightSmooth < 2 && curHeight < 0.1
    |     curHeight_correct = heightSmooth - 1.2*veld_cmd*SampeTime;
    |     if curHeight_correct < 0
    |         curHeight_correct = 0;
    |     end
    | end
    | % if heightSmooth < 2 && curHeight < 1
    | %     errHeight = heightSmooth - curHeight;
    | %     if errHeight > maxHeightVel*SampeTime
    | %         curHeight_correct = heightSmooth - maxHeightVel*SampeTime;
    | %     elseif errHeight < -maxHeightVel*SampeTime
    | %         %         curHeight_correct = heightSmooth + maxHeightVel*Ts;
    | %     end
    | % end
    | kSmooth = 0;
    | heightSmooth = kSmooth*heightSmooth + (1-kSmooth)*curHeight_correct;
    | 
    | preHeight = curHeight;
    | if heightSmooth < 0
    |     heightSmooth = 0;
    | end
    | y = heightSmooth;
  function du_func_cmd:
    | function du_func_cmd
    | persistent p_mavlink_msg_id_command_long mavCmd76UpdateCount RevNothingDuration
    | if isempty(p_mavlink_msg_id_command_long)
    |     p_mavlink_msg_id_command_long = IN_MAV.mavlink_msg_id_command_long;
    |     mavCmd76UpdateCount = IN_MAV.mav_command_long_recvflag;
    |     RevNothingDuration = 0;
    |     printComInfo('Init Cmd ID %.0f',0,p_mavlink_msg_id_command_long.command)
    | end
    | 
    | % 更新接收Cmd
    | % mavCmdChangFlag = isCmdChanged(p_mavlink_msg_id_command_long,mavlink_msg_id_command_long);
    | mavCmdChangFlag = (mavCmd76UpdateCount ~= IN_MAV.mav_command_long_recvflag);
    | mavCmd76UpdateCount = IN_MAV.mav_command_long_recvflag;
    | if mavCmdChangFlag % || mav_command_long_recvflag
    |     printComInfo('Recevie Cmd ID %.0f',0,IN_MAV.mavlink_msg_id_command_long.command)
    |     p_mavlink_msg_id_command_long = IN_MAV.mavlink_msg_id_command_long;
    |     RTInfo.Task = ENUM_RTInfo_Task.TaskLog_Mav_CmdChange; % 更新RTInfo Task 
    |     updateLogDataBuffer(ENUM_TaskLogBlockName.TASKLOG_ParserCmd,RTInfo.Task,'write'); % 更新log缓存
    |     switch IN_MAV.mavlink_msg_id_command_long.command
    |         case 241 % 航前校准 MAV_CMD_PREFLIGHT_CALIBRATION
    |             printComInfo('Cmd ID %.0f Not Response',0,p_mavlink_msg_id_command_long.command)
    |         case 20 % 返航 MAV_CMD_NAV_RETURN_TO_LAUNCH
    |             if IN_MAV.mavlink_msg_id_command_long.param1 == 0 && PathModeOut.flightTaskMode ~= ENUM_FlightTaskMode.GoHomeMode
    |                 RTInfo.GSCmd = ENUM_RTInfo_GSCmd.Recive_GoHome; % 更新RT信息
    |                 RTInfo.Task = ENUM_RTInfo_Task.TaskLog_Mav_GoHome_Yes;% 更新RTInfo Task
    |                 updateLogDataBuffer(ENUM_TaskLogBlockName.TASKLOG_ParserCmd,RTInfo.Task,'write'); % 更新log缓存
    |                 PathModeOut.typeAutoMode = ENUM_AutoModeType.SuspendTaskToHomeThenLand;
    |                 send(event_oneKeyGoHome,FLIGHTMODE.AUTO_TASK);
    |                 printComInfo('Cmd ID %.0f Response',0,p_mavlink_msg_id_command_long.command)
    |             else
    |                 RTInfo.Task = ENUM_RTInfo_Task.TaskLog_Mav_GoHome_No;% 更新RTInfo Task
    |                 updateLogDataBuffer(ENUM_TaskLogBlockName.TASKLOG_ParserCmd,RTInfo.Task,'write'); % 更新log缓存                
    |                 printComInfo('Cmd ID %.0f Not Response',0,p_mavlink_msg_id_command_long.command)
    |                 RTInfo.GSCmd = ENUM_RTInfo_GSCmd.Recive_GoHome_But_Not_Response; % 更新RT信息
    |             end
    |         case 23 % 起飞 MAV_CMD_TAKEOFF: 飞机在地面时才能激活
    |             if TaskParam.runSingleTaskMode == ENUM_FlightTaskMode.NoneFlightTaskMode % 单模式调试未激活
    |                 if IN_MAV.mavlink_msg_id_command_long.param1 == 0 && PathModeOut.whereIsUAV == ENUM_Where.OnGround && PathModeOut.flightTaskMode ~= ENUM_FlightTaskMode.TakeOffMode
    |                     RTInfo.GSCmd = ENUM_RTInfo_GSCmd.Recive_TakeOff; % 更新RT信息
    |                     RTInfo.Task = ENUM_RTInfo_Task.TaskLog_Mav_TakeOff_Yes;% 更新RTInfo Task
    |                     updateLogDataBuffer(ENUM_TaskLogBlockName.TASKLOG_ParserCmd,RTInfo.Task,'write'); % 更新log缓存                       
    |                     PathModeOut.typeAutoMode = ENUM_AutoModeType.AutoProfile; % 应对Rotor2Fix，延迟响应返航指令
    |                     send(manual_takeOff,FLIGHTMODE.AUTO_TASK);
    |                     printComInfo('Cmd ID %.0f Response',0,p_mavlink_msg_id_command_long.command)
    |                 else
    |                     RTInfo.Task = ENUM_RTInfo_Task.TaskLog_Mav_TakeOff_No; % 更新RTInfo Task
    |                     updateLogDataBuffer(ENUM_TaskLogBlockName.TASKLOG_ParserCmd,RTInfo.Task,'write'); % 更新log缓存                        
    |                     printComInfo('Cmd ID %.0f Not Response',0,p_mavlink_msg_id_command_long.command)
    |                     RTInfo.GSCmd = ENUM_RTInfo_GSCmd.Recive_TakeOff_But_Not_Response; % 更新RT信息
    |                 end
    |             end
    |         case 28 % 暂停悬停 MAV_CMD_HOVER=28
    |             if IN_MAV.mavlink_msg_id_command_long.param1 == 0 && PathModeOut.flightTaskMode ~= ENUM_FlightTaskMode.HoverAdjustMode && ...
    |                     PathModeOut.flightTaskMode ~= ENUM_FlightTaskMode.AirStandByMode
    |                 %                 PathModeOut.typeAutoMode = ENUM_AutoModeType.AutoProfile;
    |                 RTInfo.Task = ENUM_RTInfo_Task.TaskLog_Mav_HoverAdjust_Yes; % 更新RTInfo Task
    |                 updateLogDataBuffer(ENUM_TaskLogBlockName.TASKLOG_ParserCmd,RTInfo.Task,'write'); % 更新log缓存
    |                 RTInfo.GSCmd = ENUM_RTInfo_GSCmd.Recive_Pause; % 更新RT信息
    |                 send(manual_airStandBy,FLIGHTMODE.AUTO_TASK);
    |                 printComInfo('Cmd ID %.0f Response',0,p_mavlink_msg_id_command_long.command)
    |             else
    |                 RTInfo.Task = ENUM_RTInfo_Task.TaskLog_Mav_HoverAdjust_No; % 更新RTInfo Task
    |                 updateLogDataBuffer(ENUM_TaskLogBlockName.TASKLOG_ParserCmd,RTInfo.Task,'write'); % 更新log缓存                
    |                 RTInfo.GSCmd = ENUM_RTInfo_GSCmd.Recive_Pause_But_Not_Response; % 更新RT信息
    |                 printComInfo('Cmd ID %.0f Not Response',0,p_mavlink_msg_id_command_long.command)
    |             end
    |         case 29 % 继续 MAV_CMD_CONTINUE=29
    |             if ~hasTaskStarted_globalbar % 第一次点击开始任务按钮
    |                 if isPathDataValid()
    |                     RTInfo.Task = ENUM_RTInfo_Task.TaskLog_Mav_StartTask_Yes; % 更新RTInfo Task
    |                     updateLogDataBuffer(ENUM_TaskLogBlockName.TASKLOG_ParserCmd,RTInfo.Task,'write'); % 更新log缓存                           
    |                     RTInfo.GSCmd = ENUM_RTInfo_GSCmd.Recive_StartTask; % 更新RT信息
    |                     isContinuePath = false;
    |                     if PathModeOut.typeAutoMode ~= ENUM_AutoModeType.SingleModeRun
    |                         PathModeOut.typeAutoMode = ENUM_AutoModeType.AutoProfile;
    |                     end
    |                     send(event_startTaskFromAir,FLIGHTMODE.AUTO_TASK);
    |                     printComInfo('Cmd ID %.0f Start Response',0,p_mavlink_msg_id_command_long.command)
    |                 else
    |                     RTInfo.Task = ENUM_RTInfo_Task.TaskLog_Mav_StartTask_No; % 更新RTInfo Task
    |                     updateLogDataBuffer(ENUM_TaskLogBlockName.TASKLOG_ParserCmd,RTInfo.Task,'write'); % 更新log缓存                                 
    |                     RTInfo.GSCmd = ENUM_RTInfo_GSCmd.Recive_StartTask_But_Not_Response; % 更新RT信息
    |                     printComInfo('Cmd ID %.0f Start Not Response',0,p_mavlink_msg_id_command_long.command)
    |                 end
    |             else
    |                 if IN_MAV.mavlink_msg_id_command_long.param1 == 0
    |                     RTInfo.Task = ENUM_RTInfo_Task.TaskLog_Mav_Continue_Yes; % 更新RTInfo Task
    |                     updateLogDataBuffer(ENUM_TaskLogBlockName.TASKLOG_ParserCmd,RTInfo.Task,'write'); % 更新log缓存                         
    |                     RTInfo.GSCmd = ENUM_RTInfo_GSCmd.Recive_Continue; % 更新RT信息
    |                     isContinuePath = true;
    | %                     PathModeOut.typeAutoMode = ENUM_AutoModeType.AutoProfile;
    |                     send(manual_continueProfile,FLIGHTMODE.AUTO_TASK);
    |                     printComInfo('Cmd ID %.0f Continue Response',0,p_mavlink_msg_id_command_long.command)
    |                 else
    |                     RTInfo.Task = ENUM_RTInfo_Task.TaskLog_Mav_Continue_No; % 更新RTInfo Task
    |                     updateLogDataBuffer(ENUM_TaskLogBlockName.TASKLOG_ParserCmd,RTInfo.Task,'write'); % 更新log缓存                        
    |                     RTInfo.GSCmd = ENUM_RTInfo_GSCmd.Recive_Continue_But_Not_Response; % 更新RT信息
    |                     printComInfo('Cmd ID %.0f Continue Not Response',0,p_mavlink_msg_id_command_long.command)
    |                 end
    |             end
    |         case 30 % 云台检测 MAV_CMD_GIMBAL_CHECK
    |         case 31 % POS检测 MAV_CMD_POS_CHECK
    |         case 32 % 取消低电返航 MAV_CMD_CANCEL_LOWPOWER_RETURN
    |         case 33 % 取消低电降落 MAV_CMD_CANCEL_LOWPOWER_LANDING
    | %         case 34 % 倾转机构检查 MAV_CMD_Q_CHECK
    |         case 35 % 舵面检查 MAV_CMD_Q_CHECK
    |         case 36 % 切换高度 MAV_CMD_SWITCH_ALTITUDE
    |             if IN_MAV.mavlink_msg_id_command_long.param1 >= 5 % 设置保护
    |                 if PathModeOut.flightTaskMode == ENUM_FlightTaskMode.PathFollowMode || ...
    |                         PathModeOut.flightTaskMode == ENUM_FlightTaskMode.HoverUpMode
    |                     doHeightCmdKeepAfterHeightSwitch = true;
    |                 end
    |                 RTInfo.Task = ENUM_RTInfo_Task.TaskLog_Mav_SwitchHeight_Yes; % 更新RTInfo Task
    |                 updateLogDataBuffer(ENUM_TaskLogBlockName.TASKLOG_ParserCmd,RTInfo.Task,'write'); % 更新log缓存
    |                 RTInfo.GSCmd = ENUM_RTInfo_GSCmd.Recive_SwitchHeight; % 更新RT信息
    |                 CmdParam_altitude = double(IN_MAV.mavlink_msg_id_command_long.param1);
    |                 send(manual_switchHeight,FLIGHTMODE.AUTO_TASK);
    |                 printComInfo('Cmd ID %.0f Response',0,p_mavlink_msg_id_command_long.command)
    |             else
    |                 RTInfo.Task = ENUM_RTInfo_Task.TaskLog_Mav_SwitchHeight_No; % 更新RTInfo Task
    |                 updateLogDataBuffer(ENUM_TaskLogBlockName.TASKLOG_ParserCmd,RTInfo.Task,'write'); % 更新log缓存                
    |                 RTInfo.GSCmd = ENUM_RTInfo_GSCmd.Recive_SwitchHeight_But_Not_Response; % 更新RT信息
    |                 printComInfo('Cmd ID %.0f Not Response',0,p_mavlink_msg_id_command_long.command)
    |             end
    |         case 38 % 固定翼 to 多旋翼
    |             if IN_MAV.mavlink_msg_id_command_long.param1 == 1 % 设置保护
    |                 RTInfo.Task = ENUM_RTInfo_Task.TaskLog_Mav_Fix2Rotor_Yes; % 更新RTInfo Task
    |                 updateLogDataBuffer(ENUM_TaskLogBlockName.TASKLOG_ParserCmd,RTInfo.Task,'write'); % 更新log缓存                       
    |                 RTInfo.GSCmd = ENUM_RTInfo_GSCmd.Recive_Fix2Rotor; % 更新RT信息
    |                 isContinuePath = false;
    |                 PathModeOut.typeAutoMode = ENUM_AutoModeType.Fix2Rotor2HoverAdjust;
    |                 send(manual_fix2Rotor,FLIGHTMODE.AUTO_TASK);
    |                 printComInfo('Cmd ID %.0f Response',0,p_mavlink_msg_id_command_long.command)
    |             else
    |                 RTInfo.Task = ENUM_RTInfo_Task.TaskLog_Mav_Fix2Rotor_No; % 更新RTInfo Task
    |                 updateLogDataBuffer(ENUM_TaskLogBlockName.TASKLOG_ParserCmd,RTInfo.Task,'write'); % 更新log缓存                      
    |                 RTInfo.GSCmd = ENUM_RTInfo_GSCmd.Recive_Fix2Rotor_But_Not_Response; % 更新RT信息
    |                 printComInfo('Cmd ID %.0f Not Response',0,p_mavlink_msg_id_command_long.command)
    |             end
    |         case 189 % 降落 MAV_CMD_DO_LAND_START
    |             if IN_MAV.mavlink_msg_id_command_long.param1 == 1 && PathModeOut.flightTaskMode ~= ENUM_FlightTaskMode.LandMode
    | %                 PathModeOut.typeAutoMode = ENUM_AutoModeType.AutoProfile;
    |                 RTInfo.Task = ENUM_RTInfo_Task.TaskLog_Mav_Land_Yes; % 更新RTInfo Task
    |                 updateLogDataBuffer(ENUM_TaskLogBlockName.TASKLOG_ParserCmd,RTInfo.Task,'write'); % 更新log缓存           
    |                 RTInfo.GSCmd = ENUM_RTInfo_GSCmd.Recive_Land; % 更新RT信息
    |                 send(event_land_GScommand,FLIGHTMODE.AUTO_TASK);
    |                 printComInfo('Cmd ID %.0f Response',0,p_mavlink_msg_id_command_long.command)
    |             else
    |                 RTInfo.Task = ENUM_RTInfo_Task.TaskLog_Mav_Land_No; % 更新RTInfo Task
    |                 updateLogDataBuffer(ENUM_TaskLogBlockName.TASKLOG_ParserCmd,RTInfo.Task,'write'); % 更新log缓存                    
    |                 RTInfo.GSCmd = ENUM_RTInfo_GSCmd.Recive_Land_But_Not_Response; % 更新RT信息
    |                 printComInfo('Cmd ID %.0f Not Response',0,p_mavlink_msg_id_command_long.command)
    |             end
    |         case 206 % 相机触发距离 MAV_CMD_DO_SET_CAM_TRIGG_DIST
    |             if CmdParam_cameraTrigDist >= 0
    |                 RTInfo.Task = ENUM_RTInfo_Task.TaskLog_Mav_CamTrigDist_Yes; % 更新RTInfo Task
    |                 updateLogDataBuffer(ENUM_TaskLogBlockName.TASKLOG_ParserCmd,RTInfo.Task,'write'); % 更新log缓存
    |                 RTInfo.GSCmd = ENUM_RTInfo_GSCmd.Recive_CameraDist; % 更新RT信息
    |                 CmdParam_cameraTrigDist =  double(IN_MAV.mavlink_msg_id_command_long.param1);
    |                 printComInfo('Cmd ID %.0f Response',0,p_mavlink_msg_id_command_long.command)
    |             else
    |                 RTInfo.GSCmd = ENUM_RTInfo_GSCmd.Recive_CameraDist_But_Not_Response; % 更新RT信息
    |             end
    |         case 246 % 关机重启 MAV_CMD_PREFLIGHT_REBOOT_SHUTDOWN
    |         case 300 % 全过程自动任务飞行: 飞机在地面时才能激活
    |             if ~hasTaskStarted_globalbar % 第一次点击开始任务按钮
    |                 if isPathDataValid() && PathModeOut.whereIsUAV == ENUM_Where.OnGround
    |                     isContinuePath = false;
    |                     PathModeOut.typeAutoMode = ENUM_AutoModeType.AutoProfile;
    |                     send(manual_takeOff,FLIGHTMODE.AUTO_TASK);
    |                     printComInfo('Cmd ID %.0f Response',0,p_mavlink_msg_id_command_long.command)
    |                 else
    |                     printComInfo('Cmd ID %.0f Not Response',0,p_mavlink_msg_id_command_long.command)
    |                 end
    |             else
    |                 if IN_MAV.mavlink_msg_id_command_long.param1 == 0
    |                     isContinuePath = true;
    |                     PathModeOut.typeAutoMode = ENUM_AutoModeType.AutoProfile;
    |                     send(manual_continueProfile,FLIGHTMODE.AUTO_TASK);
    |                     printComInfo('Cmd ID %.0f Response',0,p_mavlink_msg_id_command_long.command)
    |                 else
    |                     printComInfo('Cmd ID %.0f Not Response',0,p_mavlink_msg_id_command_long.command)
    |                 end
    |             end
    |         case 400 % 加解锁 MAV_CMD_COMPONENT_ARM_DISARM
    |         case 267 % 工厂控制 MAV_CMD_FACTORY_CTRL
    |         case 1001 % 自定义: 进入航线模式
    |             if isPathDataValid
    |                 isContinuePath = false;
    |                 PathModeOut.typeAutoMode = ENUM_AutoModeType.NotAutoMode;
    |                 send(manual_goIntoPath,FLIGHTMODE.AUTO_TASK);
    |                 printComInfo('Cmd ID %.0f Response',0,p_mavlink_msg_id_command_long.command)
    |             end
    |         case 1003 % 自定义: 继续航线模式
    |             if isPathDataValid
    |                 isContinuePath = true;
    |                 PathModeOut.typeAutoMode = ENUM_AutoModeType.AutoProfile;
    |                 send(manual_continueProfile,FLIGHTMODE.AUTO_TASK);
    |                 printComInfo('Cmd ID %.0f Response',0,p_mavlink_msg_id_command_long.command)
    |             end
    |         case 1004 % 自定义: 定点悬停调整
    |             PathModeOut.typeAutoMode = ENUM_AutoModeType.NotAutoMode;
    |             send(manual_hoverAdjust,FLIGHTMODE.AUTO_TASK);
    |             printComInfo('Cmd ID %.0f Response',0,p_mavlink_msg_id_command_long.command)
    |         case uint8(ENUM_MavlinkStandardCmd.MavCmd_EnterGroundStandby) % 自定义: 地面待命
    |             RTInfo.Task = ENUM_RTInfo_Task.TaskLog_Mav_GroundStandby_Yes; % 更新RTInfo Task
    |             updateLogDataBuffer(ENUM_TaskLogBlockName.TASKLOG_ParserCmd,RTInfo.Task,'write'); % 更新log缓存
    |             PathModeOut.typeAutoMode = ENUM_AutoModeType.AutoProfile;
    |             if 0
    |                 send(manual_groundStandBy,FLIGHTMODE.AUTO_TASK);
    |             end
    |             printComInfo('Cmd ID %.0f Response',0,p_mavlink_msg_id_command_long.command)
    |             %                 send(manual_takeOff,FLIGHTMODE.AUTO_TASK);
    |         otherwise 
    |             sl = 1;
    |     end
    | end
    | % 重置GSCmd，由于log周期较数据周期长，为了防止有效信息丢失，延迟进行重置
    | if mavCmdChangFlag  
    |     RevNothingDuration = 0;
    | else
    |     RevNothingDuration = RevNothingDuration + 1;
    |     if RevNothingDuration > 10
    |         RTInfo.GSCmd = ENUM_RTInfo_GSCmd.Recive_Nothing; % 更新RT信息
    |     end
    | end
    | function flag = isCmdChanged(preCmdStruct,newCmdStruct)
    | flag = false;
    | if preCmdStruct.param1 ~= newCmdStruct.param1 || ...
    |         preCmdStruct.param2 ~= newCmdStruct.param2 || ...
    |         preCmdStruct.command ~= newCmdStruct.command
    |     flag = true;
    | end
  function du_func_singleMode:
    | function du_func_singleMode
    | persistent p_runSingleTaskMode
    | if isempty(p_runSingleTaskMode)
    |     p_runSingleTaskMode = TaskParam.runSingleTaskMode;
    | end
    | % 判断模式是否改变
    | isModeChanged = p_runSingleTaskMode ~= TaskParam.runSingleTaskMode;
    | if isModeChanged && TaskParam.runSingleTaskMode == ENUM_FlightTaskMode.StallRecovery
    |     send(event_stallRecovery,FLIGHTMODE.AUTO_TASK);
    | else
    |     if isModeChanged
    |         if TaskParam.runSingleTaskMode ~= ENUM_FlightTaskMode.NoneFlightTaskMode
    |             PathModeOut.typeAutoMode = ENUM_AutoModeType.SingleModeRun;
    |         end
    |         printComInfo('SingleMode %.0f',0,TaskParam.runSingleTaskMode);
    |         RTInfo.Task = ENUM_RTInfo_Task.SingleMode_Change; % 更新RTInfo Task
    |         updateLogDataBuffer(ENUM_TaskLogBlockName.TASKLOG_ParserCmd,RTInfo.Task,'write',[double(TaskParam.runSingleTaskMode);0;0;0;0]); % 更新log缓存
    |         switch TaskParam.runSingleTaskMode
    |             case ENUM_FlightTaskMode.GroundStandByMode % 地面模式
    |                 if isUavInRotor && ComFlightOut.curLLA(3) < 0.5
    |                     send(event_single_groundMode,FLIGHTMODE.AUTO_TASK);
    |                 end
    |             case ENUM_FlightTaskMode.TakeOffMode % 起飞模式
    |                 if isUavInRotor
    |                     send(event_single_takeOffMode,FLIGHTMODE.AUTO_TASK);
    |                 end
    |             case ENUM_FlightTaskMode.HoverAdjustMode % 旋翼悬停模式
    |                 if isUavInRotor
    |                     send(event_single_hoverAdjustMode,FLIGHTMODE.AUTO_TASK);
    |                 end
    |             case ENUM_FlightTaskMode.Rotor2Fix_Mode % 旋翼转固定翼模式
    |                 if isUavInRotor
    |                     send(event_single_rotor2FixMode,FLIGHTMODE.AUTO_TASK);
    |                 end
    |             case ENUM_FlightTaskMode.HoverUpMode % 盘旋上升
    |                 if isUavInFix
    |                     send(event_single_hoverUpMode,FLIGHTMODE.AUTO_TASK);
    |                 end
    |             case ENUM_FlightTaskMode.PathFollowMode
    | %                 if isUavInFix
    | %                     send(event_single_pathMode,FLIGHTMODE.AUTO_TASK);
    | %                 end
    |             case ENUM_FlightTaskMode.GoHomeMode
    | %                 send(event_single_goHomeMode,FLIGHTMODE.AUTO_TASK);
    |             case ENUM_FlightTaskMode.HoverDownMode
    | %                 if isUavInFix
    | %                     send(event_single_hoverDownMode,FLIGHTMODE.AUTO_TASK);
    | %                 end
    |             case ENUM_FlightTaskMode.Fix2Rotor_Mode
    | %                 if isUavInFix
    | %                     send(event_single_fix2RotorMode,FLIGHTMODE.AUTO_TASK);
    | %                 end
    |             case ENUM_FlightTaskMode.LandMode
    | %                 if isUavInRotor
    | %                     send(event_single_landMode,FLIGHTMODE.AUTO_TASK);
    | %                 end
    |             case ENUM_FlightTaskMode.StallRecovery
    | %                 if isUavInFix
    | %                     send(event_single_stallRecoveryMode,FLIGHTMODE.AUTO_TASK);
    | %                 end
    |             case ENUM_FlightTaskMode.VerticalMove
    |                 %             if isUavInFix
    |                 %                 send(event_single_stallRecoveryMode,FLIGHTMODE.AUTO_TASK);
    |                 %             end
    |         end
    |     end
    | end
    | p_runSingleTaskMode = TaskParam.runSingleTaskMode;
  function manual_du_func:
    | function manual_du_func
    | isAutoMode_globalvar = false;
    | % if AlgoParams.getOutOfRemote
    | %     isAutoMode_globalvar = true; % 去掉遥控器
    | % end
    | if isDebugInfoToShow
    |     fprintf('\t time %.2f [sec]: Receive Cmd: Switch to Manual!\n',clock_sec);
    | end
  function auto_du_func:
    | function auto_du_func
    | isAutoMode_globalvar = true;
    | if isDebugInfoToShow
    |     fprintf('\t time %.2f [sec]: Receive Cmd: Switch to Auto!\n',clock_sec);
    | end
  function flag = isUavInRotor:
    | function flag = isUavInRotor
    | flag = false;
    | if PathModeOut.uavMode == ENUM_UAVMode.Rotor
    |     flag = true;
    | end
  function flag = isRemoteConnected:
    | function flag = isRemoteConnected
    | persistent lostDuration
    | if isempty(lostDuration)
    |     lostDuration = 0;
    | end
    | % 遥控连接判断
    | flag = false;
    | if IN_OnPlane.isRemoteConnected
    | %     lostDuration = lostDuration + Ts;
    |     %     if lostDuration > 5 % sec
    |     %         flag = true;
    |     %     end
    |     flag = true;
    | end
    | %% 始终认为遥控器处于连接状态 V1000测试阶段之后弃用自动模式下的遥控器失联
    | if 1
    |     flag = true;
    | end
  function flag = isInTheAir:
    | function flag = isInTheAir
    | flag = false;
    | if PathModeOut.whereIsUAV == ENUM_Where.InTheAir
    |     flag = true;
    | end
  function flag = isStationConnected:
    | function flag = isStationConnected
    | persistent lostDuration
    | if isempty(lostDuration)
    |     lostDuration = 0;
    | end
    | % 遥控连接判断
    | flag = false;
    | if IN_OnPlane.isStationConnected
    |     lostDuration = lostDuration + Ts;
    | %     if lostDuration > IN_OnPlane.stationLostTimeSec % sec
    | %         flag = true;
    | %     end    
    |     flag = true;
    | end
  function en_func:
    | function en_func
    | if ~PathModeOut.isTaskComplete
    |     printDebugInfo('BreakRecord','Yes')
    |     RTInfo.Task = ENUM_RTInfo_Task.BreakRecord_Yes; % 更新RT信息
    |     updateLogDataBuffer(ENUM_TaskLogBlockName.TASKLOG_FlightMode,RTInfo.Task,'write'); % 更新log缓存
    |     PathModeOut.isNeedToRecordBreak = true;
    | end
  function du_func:
    | function du_func
    | 
    | BatteryOut.PowerConsume.AllTheTimeVoltage = double(IN_MAV.mavlink_msg_mission_current(1).voltage);
    | BatteryOut.PowerConsume.AllTheTimeCurrent = double(IN_MAV.mavlink_msg_mission_current(1).current);
    | batteryPer = double(IN_MAV.mavlink_msg_mission_current(1).remaining);
    | 
    | BatteryOut.PowerConsume.GroundStandby = 0;
    | BatteryOut.PowerConsume.TakeOff = 0;
    | BatteryOut.PowerConsume.HoverAdjust = 0;
    | BatteryOut.PowerConsume.Rotor2fix = 0;
    | BatteryOut.PowerConsume.HoverUp = 0;
    | BatteryOut.PowerConsume.PathFollow = 0;
    | BatteryOut.PowerConsume.GoHome = 0;
    | BatteryOut.PowerConsume.HoverDown = 0;
    | BatteryOut.PowerConsume.Fix2Rotor = 0;
    | BatteryOut.PowerConsume.Land = 0;
    | switch PathModeOut.flightTaskMode
    |     case ENUM_FlightTaskMode.GroundStandByMode
    |         BatteryOut.PowerConsume.GroundStandby = batteryPer;    
    |     case ENUM_FlightTaskMode.TakeOffMode
    |         BatteryOut.PowerConsume.TakeOff = batteryPer;
    |     case ENUM_FlightTaskMode.HoverAdjustMode
    |         BatteryOut.PowerConsume.HoverAdjust = batteryPer;
    |     case ENUM_FlightTaskMode.Rotor2Fix_Mode
    |         BatteryOut.PowerConsume.Rotor2fix = batteryPer;
    |     case ENUM_FlightTaskMode.HoverUpMode
    |         BatteryOut.PowerConsume.HoverUp = batteryPer;
    |     case ENUM_FlightTaskMode.PathFollowMode
    |         BatteryOut.PowerConsume.PathFollow = batteryPer;
    |     case ENUM_FlightTaskMode.GoHomeMode
    |         BatteryOut.PowerConsume.GoHome = batteryPer;
    |     case ENUM_FlightTaskMode.HoverDownMode
    |         BatteryOut.PowerConsume.HoverDown = batteryPer;
    |     case ENUM_FlightTaskMode.Fix2Rotor_Mode
    |         BatteryOut.PowerConsume.Fix2Rotor = batteryPer;        
    |     case ENUM_FlightTaskMode.LandMode
    |         BatteryOut.PowerConsume.Land = batteryPer;
    |     otherwise
    | end
    | BatteryOut.PowerConsume.AllTheTimePowerConsume = batteryPer;
  function flag = isAllowedToAutoFlight:
    | function flag = isAllowedToAutoFlight
    | flag = true;
    | if IN_SignalIntegrity.SystemHealthStatus ~= ENUM_SystemHealthStatus.SystemHealth && ...
    |         IN_SignalIntegrity.SystemHealthStatus ~= ENUM_SystemHealthStatus.DontTakeOff && ...
    |         IN_SignalIntegrity.SystemHealthStatus ~= ENUM_SystemHealthStatus.NeedToReturn && ...
    |         PathModeOut.typeAutoMode ~= ENUM_AutoModeType.NotAutoMode
    |     % 处于包线飞行模式且传感器状态不health
    |     flag = false;
    | end
  function flag = isInStall:
    | function flag = isInStall
    | flag = false;
    | curAirSpeed = double(IN_SENSOR.airspeed1.airspeed_indicate);
    | if PathModeOut.typeAutoMode ~= ENUM_AutoModeType.NotAutoMode && ... % 自动模式
    |         ~isOnGround && ... % 飞机不在地面
    |         isUavInFix && ... % 固定翼模式
    |         norm(curAirSpeed) < TaskParam.enterStallAirSpeed % 用IN_SENSOR中的原始空速而不用ComFlightOut.curAirSpeed，因为某些情况下会对ComFlightOut.curAirSpeed做改变
    | %         norm(ComFlightOut.curAirSpeed) < TaskParam.enterStallAirSpeed
    |     flag = true;     
    | end
  function info_60tick:
    |  function info_60tick
    | tabspace1 = 0;
    | RTInfo.Warning = ENUM_RTInfo_Warn.Warn_Normal;
    | if IN_SignalIntegrity.SystemHealthStatus ~= ENUM_SystemHealthStatus.SystemHealth
    |     if IN_SignalIntegrity.SystemHealthStatus == ENUM_SystemHealthStatus.DontTakeOff
    |         RTInfo.Warning = ENUM_RTInfo_Warn.Warn_SensorSystem_Not_Health;
    |         printComInfo('[System Warning] SensorSystemHealthStatus DontTakeOff',tabspace1)
    |     elseif IN_SignalIntegrity.SystemHealthStatus == ENUM_SystemHealthStatus.NeedToReturn
    |         RTInfo.Warning = ENUM_RTInfo_Warn.Warn_SensorSystem_Not_Health;
    |         printComInfo('[System Warning] SensorSystemHealthStatus NeedToReturn',tabspace1)
    |     else
    |         RTInfo.Warning = ENUM_RTInfo_Warn.Warn_SensorSystem_Not_Health;
    |         printComInfo('[System Warning] SensorSystemHealthStatus Not SystemHealth',tabspace1)
    |     end
    | end
    | 
    | if ~isAutoMode_globalvar
    |     printComInfo('[System Warning] Manual Mode',tabspace1)
    | end
    | if BatteryOut.batteryStatus ~= ENUM_BatteryStatus.BatteryNormal
    |     RTInfo.Warning = ENUM_RTInfo_Warn.Warn_Battery_Not_Normal;
    |     printComInfo('[System Warning] BatteryLife Not Normal',tabspace1)
    | end
    | if isNotInFense
    |     RTInfo.Warning = ENUM_RTInfo_Warn.Warn_Not_InFense;
    |     printComInfo('[System Warning] isNotInFense',tabspace1)
    | end
    | if ~isRemoteConnected
    |     RTInfo.Warning = ENUM_RTInfo_Warn.Warn_Remote_Not_Connect;
    |     printComInfo('[System Warning] Remote Lost',tabspace1)
    | end
    | if isStationLostForAWhile
    |     RTInfo.Warning = ENUM_RTInfo_Warn.Warn_Station_Not_Connect;
    |     printComInfo('[System Warning] GroundStation Lost',tabspace1)
    | end 
    | if ~isPathDataValid
